simulink model "model_compatible"  (Simulink 7.5)
(part 3 of 4)

      | %<VLF>pu
      | %<angleLF>deg.
      | %<Name>
  bus158 : powerlib/Measurements/Load Flow Bus  LConnTagsString=a  Phases=single  Connectors=on one side  ID=bus158  Vbase=220000  Vref=1  Vangle=0  VLF=1  VLFb=1  VLFc=1  angleLF=0  angleLFb=0  angleLFc=0
      settings: AttributesFormatString=|
      | %<ID>
      | %<Vbase>V
      | %<VLF>pu
      | %<angleLF>deg.
      | %<Name>
  bus159 : powerlib/Measurements/Load Flow Bus  LConnTagsString=a  Phases=single  Connectors=on one side  ID=bus159  Vbase=220000  Vref=1  Vangle=0  VLF=1  VLFb=1  VLFc=1  angleLF=0  angleLFb=0  angleLFc=0
      settings: AttributesFormatString=|
      | %<ID>
      | %<Vbase>V
      | %<VLF>pu
      | %<angleLF>deg.
      | %<Name>
  bus16 : powerlib/Measurements/Load Flow Bus  LConnTagsString=a  Phases=single  Connectors=on one side  ID=bus16  Vbase=220000  Vref=1  Vangle=0  VLF=1  VLFb=1  VLFc=1  angleLF=0  angleLFb=0  angleLFc=0
      settings: AttributesFormatString=|
      | %<ID>
      | %<Vbase>V
      | %<VLF>pu
      | %<angleLF>deg.
      | %<Name>
  bus160 : powerlib/Measurements/Load Flow Bus  LConnTagsString=a  Phases=single  Connectors=on one side  ID=bus160  Vbase=220000  Vref=1  Vangle=0  VLF=1  VLFb=1  VLFc=1  angleLF=0  angleLFb=0  angleLFc=0
      settings: AttributesFormatString=|
      | %<ID>
      | %<Vbase>V
      | %<VLF>pu
      | %<angleLF>deg.
      | %<Name>
  bus161 : powerlib/Measurements/Load Flow Bus  LConnTagsString=a  Phases=single  Connectors=on one side  ID=bus161  Vbase=220000  Vref=1  Vangle=0  VLF=1  VLFb=1  VLFc=1  angleLF=0  angleLFb=0  angleLFc=0
      settings: AttributesFormatString=|
      | %<ID>
      | %<Vbase>V
      | %<VLF>pu
      | %<angleLF>deg.
      | %<Name>
  bus162 : powerlib/Measurements/Load Flow Bus  LConnTagsString=a  Phases=single  Connectors=on one side  ID=bus162  Vbase=220000  Vref=1  Vangle=0  VLF=1  VLFb=1  VLFc=1  angleLF=0  angleLFb=0  angleLFc=0
      settings: AttributesFormatString=|
      | %<ID>
      | %<Vbase>V
      | %<VLF>pu
      | %<angleLF>deg.
      | %<Name>
  bus163 : powerlib/Measurements/Load Flow Bus  LConnTagsString=a  Phases=single  Connectors=on one side  ID=bus163  Vbase=220000  Vref=1  Vangle=0  VLF=1  VLFb=1  VLFc=1  angleLF=0  angleLFb=0  angleLFc=0
      settings: AttributesFormatString=|
      | %<ID>
      | %<Vbase>V
      | %<VLF>pu
      | %<angleLF>deg.
      | %<Name>
  bus164 : powerlib/Measurements/Load Flow Bus  LConnTagsString=a  Phases=single  Connectors=on one side  ID=bus164  Vbase=220000  Vref=1  Vangle=0  VLF=1  VLFb=1  VLFc=1  angleLF=0  angleLFb=0  angleLFc=0
      settings: AttributesFormatString=|
      | %<ID>
      | %<Vbase>V
      | %<VLF>pu
      | %<angleLF>deg.
      | %<Name>
  bus165 : powerlib/Measurements/Load Flow Bus  LConnTagsString=a  Phases=single  Connectors=on one side  ID=bus165  Vbase=220000  Vref=1  Vangle=0  VLF=1  VLFb=1  VLFc=1  angleLF=0  angleLFb=0  angleLFc=0
      settings: AttributesFormatString=|
      | %<ID>
      | %<Vbase>V
      | %<VLF>pu
      | %<angleLF>deg.
      | %<Name>
  bus166 : powerlib/Measurements/Load Flow Bus  LConnTagsString=a  Phases=single  Connectors=on one side  ID=bus166  Vbase=220000  Vref=1  Vangle=0  VLF=1  VLFb=1  VLFc=1  angleLF=0  angleLFb=0  angleLFc=0
      settings: AttributesFormatString=|
      | %<ID>
      | %<Vbase>V
      | %<VLF>pu
      | %<angleLF>deg.
      | %<Name>
  bus167 : powerlib/Measurements/Load Flow Bus  LConnTagsString=a  Phases=single  Connectors=on one side  ID=bus167  Vbase=220000  Vref=1  Vangle=0  VLF=1  VLFb=1  VLFc=1  angleLF=0  angleLFb=0  angleLFc=0
      settings: AttributesFormatString=|
      | %<ID>
      | %<Vbase>V
      | %<VLF>pu
      | %<angleLF>deg.
      | %<Name>
  bus168 : powerlib/Measurements/Load Flow Bus  LConnTagsString=a  Phases=single  Connectors=on one side  ID=bus168  Vbase=220000  Vref=1  Vangle=0  VLF=1  VLFb=1  VLFc=1  angleLF=0  angleLFb=0  angleLFc=0
      settings: AttributesFormatString=|
      | %<ID>
      | %<Vbase>V
      | %<VLF>pu
      | %<angleLF>deg.
      | %<Name>
  bus169 : powerlib/Measurements/Load Flow Bus  LConnTagsString=a  Phases=single  Connectors=on one side  ID=bus169  Vbase=220000  Vref=1  Vangle=0  VLF=1  VLFb=1  VLFc=1  angleLF=0  angleLFb=0  angleLFc=0
      settings: AttributesFormatString=|
      | %<ID>
      | %<Vbase>V
      | %<VLF>pu
      | %<angleLF>deg.
      | %<Name>
  bus17 : powerlib/Measurements/Load Flow Bus  LConnTagsString=a  Phases=single  Connectors=on one side  ID=bus17  Vbase=220000  Vref=1  Vangle=0  VLF=1  VLFb=1  VLFc=1  angleLF=0  angleLFb=0  angleLFc=0
      settings: AttributesFormatString=|
      | %<ID>
      | %<Vbase>V
      | %<VLF>pu
      | %<angleLF>deg.
      | %<Name>
  bus170 : powerlib/Measurements/Load Flow Bus  LConnTagsString=a  Phases=single  Connectors=on one side  ID=bus170  Vbase=220000  Vref=1  Vangle=0  VLF=1  VLFb=1  VLFc=1  angleLF=0  angleLFb=0  angleLFc=0
      settings: AttributesFormatString=|
      | %<ID>
      | %<Vbase>V
      | %<VLF>pu
      | %<angleLF>deg.
      | %<Name>
  bus171 : powerlib/Measurements/Load Flow Bus  LConnTagsString=a  Phases=single  Connectors=on one side  ID=bus171  Vbase=220000  Vref=1  Vangle=0  VLF=1  VLFb=1  VLFc=1  angleLF=0  angleLFb=0  angleLFc=0
      settings: AttributesFormatString=|
      | %<ID>
      | %<Vbase>V
      | %<VLF>pu
      | %<angleLF>deg.
      | %<Name>
  bus172 : powerlib/Measurements/Load Flow Bus  LConnTagsString=a  Phases=single  Connectors=on one side  ID=bus172  Vbase=220000  Vref=1  Vangle=0  VLF=1  VLFb=1  VLFc=1  angleLF=0  angleLFb=0  angleLFc=0
      settings: AttributesFormatString=|
      | %<ID>
      | %<Vbase>V
      | %<VLF>pu
      | %<angleLF>deg.
      | %<Name>
  bus173 : powerlib/Measurements/Load Flow Bus  LConnTagsString=a  Phases=single  Connectors=on one side  ID=bus173  Vbase=220000  Vref=1  Vangle=0  VLF=1  VLFb=1  VLFc=1  angleLF=0  angleLFb=0  angleLFc=0
      settings: AttributesFormatString=|
      | %<ID>
      | %<Vbase>V
      | %<VLF>pu
      | %<angleLF>deg.
      | %<Name>
  bus174 : powerlib/Measurements/Load Flow Bus  LConnTagsString=a  Phases=single  Connectors=on one side  ID=bus174  Vbase=220000  Vref=1  Vangle=0  VLF=1  VLFb=1  VLFc=1  angleLF=0  angleLFb=0  angleLFc=0
      settings: AttributesFormatString=|
      | %<ID>
      | %<Vbase>V
      | %<VLF>pu
      | %<angleLF>deg.
      | %<Name>
  bus175 : powerlib/Measurements/Load Flow Bus  LConnTagsString=a  Phases=single  Connectors=on one side  ID=bus175  Vbase=220000  Vref=1  Vangle=0  VLF=1  VLFb=1  VLFc=1  angleLF=0  angleLFb=0  angleLFc=0
      settings: AttributesFormatString=|
      | %<ID>
      | %<Vbase>V
      | %<VLF>pu
      | %<angleLF>deg.
      | %<Name>
  bus176 : powerlib/Measurements/Load Flow Bus  LConnTagsString=a  Phases=single  Connectors=on one side  ID=bus176  Vbase=220000  Vref=1  Vangle=0  VLF=1  VLFb=1  VLFc=1  angleLF=0  angleLFb=0  angleLFc=0
      settings: AttributesFormatString=|
      | %<ID>
      | %<Vbase>V
      | %<VLF>pu
      | %<angleLF>deg.
      | %<Name>
  bus177 : powerlib/Measurements/Load Flow Bus  LConnTagsString=a  Phases=single  Connectors=on one side  ID=bus177  Vbase=220000  Vref=1  Vangle=0  VLF=1  VLFb=1  VLFc=1  angleLF=0  angleLFb=0  angleLFc=0
      settings: AttributesFormatString=|
      | %<ID>
      | %<Vbase>V
      | %<VLF>pu
      | %<angleLF>deg.
      | %<Name>
  bus178 : powerlib/Measurements/Load Flow Bus  LConnTagsString=a  Phases=single  Connectors=on one side  ID=bus178  Vbase=220000  Vref=1  Vangle=0  VLF=1  VLFb=1  VLFc=1  angleLF=0  angleLFb=0  angleLFc=0
      settings: AttributesFormatString=|
      | %<ID>
      | %<Vbase>V
      | %<VLF>pu
      | %<angleLF>deg.
      | %<Name>
  bus179 : powerlib/Measurements/Load Flow Bus  LConnTagsString=a  Phases=single  Connectors=on one side  ID=bus179  Vbase=220000  Vref=1  Vangle=0  VLF=1  VLFb=1  VLFc=1  angleLF=0  angleLFb=0  angleLFc=0
      settings: AttributesFormatString=|
      | %<ID>
      | %<Vbase>V
      | %<VLF>pu
      | %<angleLF>deg.
      | %<Name>
  bus18 : powerlib/Measurements/Load Flow Bus  LConnTagsString=a  Phases=single  Connectors=on one side  ID=bus18  Vbase=220000  Vref=1  Vangle=0  VLF=1  VLFb=1  VLFc=1  angleLF=0  angleLFb=0  angleLFc=0
      settings: AttributesFormatString=|
      | %<ID>
      | %<Vbase>V
      | %<VLF>pu
      | %<angleLF>deg.
      | %<Name>
  bus180 : powerlib/Measurements/Load Flow Bus  LConnTagsString=a  Phases=single  Connectors=on one side  ID=bus180  Vbase=220000  Vref=1  Vangle=0  VLF=1  VLFb=1  VLFc=1  angleLF=0  angleLFb=0  angleLFc=0
      settings: AttributesFormatString=|
      | %<ID>
      | %<Vbase>V
      | %<VLF>pu
      | %<angleLF>deg.
      | %<Name>
  bus181 : powerlib/Measurements/Load Flow Bus  LConnTagsString=a  Phases=single  Connectors=on one side  ID=bus181  Vbase=220000  Vref=1  Vangle=0  VLF=1  VLFb=1  VLFc=1  angleLF=0  angleLFb=0  angleLFc=0
      settings: AttributesFormatString=|
      | %<ID>
      | %<Vbase>V
      | %<VLF>pu
      | %<angleLF>deg.
      | %<Name>
  bus182 : powerlib/Measurements/Load Flow Bus  LConnTagsString=a  Phases=single  Connectors=on one side  ID=bus182  Vbase=220000  Vref=1  Vangle=0  VLF=1  VLFb=1  VLFc=1  angleLF=0  angleLFb=0  angleLFc=0
      settings: AttributesFormatString=|
      | %<ID>
      | %<Vbase>V
      | %<VLF>pu
      | %<angleLF>deg.
      | %<Name>
  bus183 : powerlib/Measurements/Load Flow Bus  LConnTagsString=a  Phases=single  Connectors=on one side  ID=bus183  Vbase=220000  Vref=1  Vangle=0  VLF=1  VLFb=1  VLFc=1  angleLF=0  angleLFb=0  angleLFc=0
      settings: AttributesFormatString=|
      | %<ID>
      | %<Vbase>V
      | %<VLF>pu
      | %<angleLF>deg.
      | %<Name>
  bus184 : powerlib/Measurements/Load Flow Bus  LConnTagsString=a  Phases=single  Connectors=on one side  ID=bus184  Vbase=220000  Vref=1  Vangle=0  VLF=1  VLFb=1  VLFc=1  angleLF=0  angleLFb=0  angleLFc=0
      settings: AttributesFormatString=|
      | %<ID>
      | %<Vbase>V
      | %<VLF>pu
      | %<angleLF>deg.
      | %<Name>
  bus185 : powerlib/Measurements/Load Flow Bus  LConnTagsString=a  Phases=single  Connectors=on one side  ID=bus185  Vbase=220000  Vref=1  Vangle=0  VLF=1  VLFb=1  VLFc=1  angleLF=0  angleLFb=0  angleLFc=0
      settings: AttributesFormatString=|
      | %<ID>
      | %<Vbase>V
      | %<VLF>pu
      | %<angleLF>deg.
      | %<Name>
  bus186 : powerlib/Measurements/Load Flow Bus  LConnTagsString=a  Phases=single  Connectors=on one side  ID=bus186  Vbase=220000  Vref=1  Vangle=0  VLF=1  VLFb=1  VLFc=1  angleLF=0  angleLFb=0  angleLFc=0
      settings: AttributesFormatString=|
      | %<ID>
      | %<Vbase>V
      | %<VLF>pu
      | %<angleLF>deg.
      | %<Name>
  bus187 : powerlib/Measurements/Load Flow Bus  LConnTagsString=a  Phases=single  Connectors=on one side  ID=bus187  Vbase=220000  Vref=1  Vangle=0  VLF=1  VLFb=1  VLFc=1  angleLF=0  angleLFb=0  angleLFc=0
      settings: AttributesFormatString=|
      | %<ID>
      | %<Vbase>V
      | %<VLF>pu
      | %<angleLF>deg.
      | %<Name>
  bus188 : powerlib/Measurements/Load Flow Bus  LConnTagsString=a  Phases=single  Connectors=on one side  ID=bus188  Vbase=220000  Vref=1  Vangle=0  VLF=1  VLFb=1  VLFc=1  angleLF=0  angleLFb=0  angleLFc=0
      settings: AttributesFormatString=|
      | %<ID>
      | %<Vbase>V
      | %<VLF>pu
      | %<angleLF>deg.
      | %<Name>
  bus189 : powerlib/Measurements/Load Flow Bus  LConnTagsString=a  Phases=single  Connectors=on one side  ID=bus189  Vbase=220000  Vref=1  Vangle=0  VLF=1  VLFb=1  VLFc=1  angleLF=0  angleLFb=0  angleLFc=0
      settings: AttributesFormatString=|
      | %<ID>
      | %<Vbase>V
      | %<VLF>pu
      | %<angleLF>deg.
      | %<Name>
  bus19 : powerlib/Measurements/Load Flow Bus  LConnTagsString=a  Phases=single  Connectors=on one side  ID=bus19  Vbase=220000  Vref=1  Vangle=0  VLF=1  VLFb=1  VLFc=1  angleLF=0  angleLFb=0  angleLFc=0
      settings: AttributesFormatString=|
      | %<ID>
      | %<Vbase>V
      | %<VLF>pu
      | %<angleLF>deg.
      | %<Name>
  bus190 : powerlib/Measurements/Load Flow Bus  LConnTagsString=a  Phases=single  Connectors=on one side  ID=bus190  Vbase=220000  Vref=1  Vangle=0  VLF=1  VLFb=1  VLFc=1  angleLF=0  angleLFb=0  angleLFc=0
      settings: AttributesFormatString=|
      | %<ID>
      | %<Vbase>V
      | %<VLF>pu
      | %<angleLF>deg.
      | %<Name>
  bus191 : powerlib/Measurements/Load Flow Bus  LConnTagsString=a  Phases=single  Connectors=on one side  ID=bus191  Vbase=220000  Vref=1  Vangle=0  VLF=1  VLFb=1  VLFc=1  angleLF=0  angleLFb=0  angleLFc=0
      settings: AttributesFormatString=|
      | %<ID>
      | %<Vbase>V
      | %<VLF>pu
      | %<angleLF>deg.
      | %<Name>
  bus192 : powerlib/Measurements/Load Flow Bus  LConnTagsString=a  Phases=single  Connectors=on one side  ID=bus192  Vbase=220000  Vref=1  Vangle=0  VLF=1  VLFb=1  VLFc=1  angleLF=0  angleLFb=0  angleLFc=0
      settings: AttributesFormatString=|
      | %<ID>
      | %<Vbase>V
      | %<VLF>pu
      | %<angleLF>deg.
      | %<Name>
  bus193 : powerlib/Measurements/Load Flow Bus  LConnTagsString=a  Phases=single  Connectors=on one side  ID=bus193  Vbase=220000  Vref=1  Vangle=0  VLF=1  VLFb=1  VLFc=1  angleLF=0  angleLFb=0  angleLFc=0
      settings: AttributesFormatString=|
      | %<ID>
      | %<Vbase>V
      | %<VLF>pu
      | %<angleLF>deg.
      | %<Name>
  bus194 : powerlib/Measurements/Load Flow Bus  LConnTagsString=a  Phases=single  Connectors=on one side  ID=bus194  Vbase=220000  Vref=1  Vangle=0  VLF=1  VLFb=1  VLFc=1  angleLF=0  angleLFb=0  angleLFc=0
      settings: AttributesFormatString=|
      | %<ID>
      | %<Vbase>V
      | %<VLF>pu
      | %<angleLF>deg.
      | %<Name>
  bus195 : powerlib/Measurements/Load Flow Bus  LConnTagsString=a  Phases=single  Connectors=on one side  ID=bus195  Vbase=220000  Vref=1  Vangle=0  VLF=1  VLFb=1  VLFc=1  angleLF=0  angleLFb=0  angleLFc=0
      settings: AttributesFormatString=|
      | %<ID>
      | %<Vbase>V
      | %<VLF>pu
      | %<angleLF>deg.
      | %<Name>
  bus196 : powerlib/Measurements/Load Flow Bus  LConnTagsString=a  Phases=single  Connectors=on one side  ID=bus196  Vbase=220000  Vref=1  Vangle=0  VLF=1  VLFb=1  VLFc=1  angleLF=0  angleLFb=0  angleLFc=0
      settings: AttributesFormatString=|
      | %<ID>
      | %<Vbase>V
      | %<VLF>pu
      | %<angleLF>deg.
      | %<Name>
  bus197 : powerlib/Measurements/Load Flow Bus  LConnTagsString=a  Phases=single  Connectors=on one side  ID=bus197  Vbase=220000  Vref=1  Vangle=0  VLF=1  VLFb=1  VLFc=1  angleLF=0  angleLFb=0  angleLFc=0
      settings: AttributesFormatString=|
      | %<ID>
      | %<Vbase>V
      | %<VLF>pu
      | %<angleLF>deg.
      | %<Name>
  bus198 : powerlib/Measurements/Load Flow Bus  LConnTagsString=a  Phases=single  Connectors=on one side  ID=bus198  Vbase=220000  Vref=1  Vangle=0  VLF=1  VLFb=1  VLFc=1  angleLF=0  angleLFb=0  angleLFc=0
      settings: AttributesFormatString=|
      | %<ID>
      | %<Vbase>V
      | %<VLF>pu
      | %<angleLF>deg.
      | %<Name>
  bus199 : powerlib/Measurements/Load Flow Bus  LConnTagsString=a  Phases=single  Connectors=on one side  ID=bus199  Vbase=220000  Vref=1  Vangle=0  VLF=1  VLFb=1  VLFc=1  angleLF=0  angleLFb=0  angleLFc=0
      settings: AttributesFormatString=|
      | %<ID>
      | %<Vbase>V
      | %<VLF>pu
      | %<angleLF>deg.
      | %<Name>
  bus2 : powerlib/Measurements/Load Flow Bus  LConnTagsString=a  Phases=single  Connectors=on one side  ID=bus2  Vbase=220000  Vref=1  Vangle=0  VLF=1  VLFb=1  VLFc=1  angleLF=0  angleLFb=0  angleLFc=0
      settings: AttributesFormatString=|
      | %<ID>
      | %<Vbase>V
      | %<VLF>pu
      | %<angleLF>deg.
      | %<Name>
  bus20 : powerlib/Measurements/Load Flow Bus  LConnTagsString=a  Phases=single  Connectors=on one side  ID=bus20  Vbase=220000  Vref=1  Vangle=0  VLF=1  VLFb=1  VLFc=1  angleLF=0  angleLFb=0  angleLFc=0
      settings: AttributesFormatString=|
      | %<ID>
      | %<Vbase>V
      | %<VLF>pu
      | %<angleLF>deg.
      | %<Name>
  bus200 : powerlib/Measurements/Load Flow Bus  LConnTagsString=a  Phases=single  Connectors=on one side  ID=bus200  Vbase=220000  Vref=1  Vangle=0  VLF=1  VLFb=1  VLFc=1  angleLF=0  angleLFb=0  angleLFc=0
      settings: AttributesFormatString=|
      | %<ID>
      | %<Vbase>V
      | %<VLF>pu
      | %<angleLF>deg.
      | %<Name>
  bus201 : powerlib/Measurements/Load Flow Bus  LConnTagsString=a  Phases=single  Connectors=on one side  ID=bus201  Vbase=220000  Vref=1  Vangle=0  VLF=1  VLFb=1  VLFc=1  angleLF=0  angleLFb=0  angleLFc=0
      settings: AttributesFormatString=|
      | %<ID>
      | %<Vbase>V
      | %<VLF>pu
      | %<angleLF>deg.
      | %<Name>
  bus202 : powerlib/Measurements/Load Flow Bus  LConnTagsString=a  Phases=single  Connectors=on one side  ID=bus202  Vbase=220000  Vref=1  Vangle=0  VLF=1  VLFb=1  VLFc=1  angleLF=0  angleLFb=0  angleLFc=0
      settings: AttributesFormatString=|
      | %<ID>
      | %<Vbase>V
      | %<VLF>pu
      | %<angleLF>deg.
      | %<Name>
  bus203 : powerlib/Measurements/Load Flow Bus  LConnTagsString=a  Phases=single  Connectors=on one side  ID=bus203  Vbase=220000  Vref=1  Vangle=0  VLF=1  VLFb=1  VLFc=1  angleLF=0  angleLFb=0  angleLFc=0
      settings: AttributesFormatString=|
      | %<ID>
      | %<Vbase>V
      | %<VLF>pu
      | %<angleLF>deg.
      | %<Name>
  bus204 : powerlib/Measurements/Load Flow Bus  LConnTagsString=a  Phases=single  Connectors=on one side  ID=bus204  Vbase=220000  Vref=1  Vangle=0  VLF=1  VLFb=1  VLFc=1  angleLF=0  angleLFb=0  angleLFc=0
      settings: AttributesFormatString=|
      | %<ID>
      | %<Vbase>V
      | %<VLF>pu
      | %<angleLF>deg.
      | %<Name>
  bus205 : powerlib/Measurements/Load Flow Bus  LConnTagsString=a  Phases=single  Connectors=on one side  ID=bus205  Vbase=220000  Vref=1  Vangle=0  VLF=1  VLFb=1  VLFc=1  angleLF=0  angleLFb=0  angleLFc=0
      settings: AttributesFormatString=|
      | %<ID>
      | %<Vbase>V
      | %<VLF>pu
      | %<angleLF>deg.
      | %<Name>
  bus206 : powerlib/Measurements/Load Flow Bus  LConnTagsString=a  Phases=single  Connectors=on one side  ID=bus206  Vbase=220000  Vref=1  Vangle=0  VLF=1  VLFb=1  VLFc=1  angleLF=0  angleLFb=0  angleLFc=0
      settings: AttributesFormatString=|
      | %<ID>
      | %<Vbase>V
      | %<VLF>pu
      | %<angleLF>deg.
      | %<Name>
  bus207 : powerlib/Measurements/Load Flow Bus  LConnTagsString=a  Phases=single  Connectors=on one side  ID=bus207  Vbase=220000  Vref=1  Vangle=0  VLF=1  VLFb=1  VLFc=1  angleLF=0  angleLFb=0  angleLFc=0
      settings: AttributesFormatString=|
      | %<ID>
      | %<Vbase>V
      | %<VLF>pu
      | %<angleLF>deg.
      | %<Name>
  bus208 : powerlib/Measurements/Load Flow Bus  LConnTagsString=a  Phases=single  Connectors=on one side  ID=bus208  Vbase=220000  Vref=1  Vangle=0  VLF=1  VLFb=1  VLFc=1  angleLF=0  angleLFb=0  angleLFc=0
      settings: AttributesFormatString=|
      | %<ID>
      | %<Vbase>V
      | %<VLF>pu
      | %<angleLF>deg.
      | %<Name>
  bus209 : powerlib/Measurements/Load Flow Bus  LConnTagsString=a  Phases=single  Connectors=on one side  ID=bus209  Vbase=220000  Vref=1  Vangle=0  VLF=1  VLFb=1  VLFc=1  angleLF=0  angleLFb=0  angleLFc=0
      settings: AttributesFormatString=|
      | %<ID>
      | %<Vbase>V
      | %<VLF>pu
      | %<angleLF>deg.
      | %<Name>
  bus21 : powerlib/Measurements/Load Flow Bus  LConnTagsString=a  Phases=single  Connectors=on one side  ID=bus21  Vbase=220000  Vref=1  Vangle=0  VLF=1  VLFb=1  VLFc=1  angleLF=0  angleLFb=0  angleLFc=0
      settings: AttributesFormatString=|
      | %<ID>
      | %<Vbase>V
      | %<VLF>pu
      | %<angleLF>deg.
      | %<Name>
  bus210 : powerlib/Measurements/Load Flow Bus  LConnTagsString=a  Phases=single  Connectors=on one side  ID=bus210  Vbase=220000  Vref=1  Vangle=0  VLF=1  VLFb=1  VLFc=1  angleLF=0  angleLFb=0  angleLFc=0
      settings: AttributesFormatString=|
      | %<ID>
      | %<Vbase>V
      | %<VLF>pu
      | %<angleLF>deg.
      | %<Name>
  bus211 : powerlib/Measurements/Load Flow Bus  LConnTagsString=a  Phases=single  Connectors=on one side  ID=bus211  Vbase=220000  Vref=1  Vangle=0  VLF=1  VLFb=1  VLFc=1  angleLF=0  angleLFb=0  angleLFc=0
      settings: AttributesFormatString=|
      | %<ID>
      | %<Vbase>V
      | %<VLF>pu
      | %<angleLF>deg.
      | %<Name>
  bus212 : powerlib/Measurements/Load Flow Bus  LConnTagsString=a  Phases=single  Connectors=on one side  ID=bus212  Vbase=220000  Vref=1  Vangle=0  VLF=1  VLFb=1  VLFc=1  angleLF=0  angleLFb=0  angleLFc=0
      settings: AttributesFormatString=|
      | %<ID>
      | %<Vbase>V
      | %<VLF>pu
      | %<angleLF>deg.
      | %<Name>
  bus213 : powerlib/Measurements/Load Flow Bus  LConnTagsString=a  Phases=single  Connectors=on one side  ID=bus213  Vbase=220000  Vref=1  Vangle=0  VLF=1  VLFb=1  VLFc=1  angleLF=0  angleLFb=0  angleLFc=0
      settings: AttributesFormatString=|
      | %<ID>
      | %<Vbase>V
      | %<VLF>pu
      | %<angleLF>deg.
      | %<Name>
  bus214 : powerlib/Measurements/Load Flow Bus  LConnTagsString=a  Phases=single  Connectors=on one side  ID=bus214  Vbase=220000  Vref=1  Vangle=0  VLF=1  VLFb=1  VLFc=1  angleLF=0  angleLFb=0  angleLFc=0
      settings: AttributesFormatString=|
      | %<ID>
      | %<Vbase>V
      | %<VLF>pu
      | %<angleLF>deg.
      | %<Name>
  bus215 : powerlib/Measurements/Load Flow Bus  LConnTagsString=a  Phases=single  Connectors=on one side  ID=bus215  Vbase=220000  Vref=1  Vangle=0  VLF=1  VLFb=1  VLFc=1  angleLF=0  angleLFb=0  angleLFc=0
      settings: AttributesFormatString=|
      | %<ID>
      | %<Vbase>V
      | %<VLF>pu
      | %<angleLF>deg.
      | %<Name>
  bus216 : powerlib/Measurements/Load Flow Bus  LConnTagsString=a  Phases=single  Connectors=on one side  ID=bus216  Vbase=220000  Vref=1  Vangle=0  VLF=1  VLFb=1  VLFc=1  angleLF=0  angleLFb=0  angleLFc=0
      settings: AttributesFormatString=|
      | %<ID>
      | %<Vbase>V
      | %<VLF>pu
      | %<angleLF>deg.
      | %<Name>
  bus217 : powerlib/Measurements/Load Flow Bus  LConnTagsString=a  Phases=single  Connectors=on one side  ID=bus217  Vbase=220000  Vref=1  Vangle=0  VLF=1  VLFb=1  VLFc=1  angleLF=0  angleLFb=0  angleLFc=0
      settings: AttributesFormatString=|
      | %<ID>
      | %<Vbase>V
      | %<VLF>pu
      | %<angleLF>deg.
      | %<Name>
  bus218 : powerlib/Measurements/Load Flow Bus  LConnTagsString=a  Phases=single  Connectors=on one side  ID=bus218  Vbase=220000  Vref=1  Vangle=0  VLF=1  VLFb=1  VLFc=1  angleLF=0  angleLFb=0  angleLFc=0
      settings: AttributesFormatString=|
      | %<ID>
      | %<Vbase>V
      | %<VLF>pu
      | %<angleLF>deg.
      | %<Name>
  bus219 : powerlib/Measurements/Load Flow Bus  LConnTagsString=a  Phases=single  Connectors=on one side  ID=bus219  Vbase=220000  Vref=1  Vangle=0  VLF=1  VLFb=1  VLFc=1  angleLF=0  angleLFb=0  angleLFc=0
      settings: AttributesFormatString=|
      | %<ID>
      | %<Vbase>V
      | %<VLF>pu
      | %<angleLF>deg.
      | %<Name>
  bus22 : powerlib/Measurements/Load Flow Bus  LConnTagsString=a  Phases=single  Connectors=on one side  ID=bus22  Vbase=220000  Vref=1  Vangle=0  VLF=1  VLFb=1  VLFc=1  angleLF=0  angleLFb=0  angleLFc=0
      settings: AttributesFormatString=|
      | %<ID>
      | %<Vbase>V
      | %<VLF>pu
      | %<angleLF>deg.
      | %<Name>
  bus220 : powerlib/Measurements/Load Flow Bus  LConnTagsString=a  Phases=single  Connectors=on one side  ID=bus220  Vbase=220000  Vref=1  Vangle=0  VLF=1  VLFb=1  VLFc=1  angleLF=0  angleLFb=0  angleLFc=0
      settings: AttributesFormatString=|
      | %<ID>
      | %<Vbase>V
      | %<VLF>pu
      | %<angleLF>deg.
      | %<Name>
  bus221 : powerlib/Measurements/Load Flow Bus  LConnTagsString=a  Phases=single  Connectors=on one side  ID=bus221  Vbase=220000  Vref=1  Vangle=0  VLF=1  VLFb=1  VLFc=1  angleLF=0  angleLFb=0  angleLFc=0
      settings: AttributesFormatString=|
      | %<ID>
      | %<Vbase>V
      | %<VLF>pu
      | %<angleLF>deg.
      | %<Name>
  bus222 : powerlib/Measurements/Load Flow Bus  LConnTagsString=a  Phases=single  Connectors=on one side  ID=bus222  Vbase=220000  Vref=1  Vangle=0  VLF=1  VLFb=1  VLFc=1  angleLF=0  angleLFb=0  angleLFc=0
      settings: AttributesFormatString=|
      | %<ID>
      | %<Vbase>V
      | %<VLF>pu
      | %<angleLF>deg.
      | %<Name>
  bus223 : powerlib/Measurements/Load Flow Bus  LConnTagsString=a  Phases=single  Connectors=on one side  ID=bus223  Vbase=220000  Vref=1  Vangle=0  VLF=1  VLFb=1  VLFc=1  angleLF=0  angleLFb=0  angleLFc=0
      settings: AttributesFormatString=|
      | %<ID>
      | %<Vbase>V
      | %<VLF>pu
      | %<angleLF>deg.
      | %<Name>
  bus224 : powerlib/Measurements/Load Flow Bus  LConnTagsString=a  Phases=single  Connectors=on one side  ID=bus224  Vbase=220000  Vref=1  Vangle=0  VLF=1  VLFb=1  VLFc=1  angleLF=0  angleLFb=0  angleLFc=0
      settings: AttributesFormatString=|
      | %<ID>
      | %<Vbase>V
      | %<VLF>pu
      | %<angleLF>deg.
      | %<Name>
  bus225 : powerlib/Measurements/Load Flow Bus  LConnTagsString=a  Phases=single  Connectors=on one side  ID=bus225  Vbase=220000  Vref=1  Vangle=0  VLF=1  VLFb=1  VLFc=1  angleLF=0  angleLFb=0  angleLFc=0
      settings: AttributesFormatString=|
      | %<ID>
      | %<Vbase>V
      | %<VLF>pu
      | %<angleLF>deg.
      | %<Name>
  bus226 : powerlib/Measurements/Load Flow Bus  LConnTagsString=a  Phases=single  Connectors=on one side  ID=bus226  Vbase=220000  Vref=1  Vangle=0  VLF=1  VLFb=1  VLFc=1  angleLF=0  angleLFb=0  angleLFc=0
      settings: AttributesFormatString=|
      | %<ID>
      | %<Vbase>V
      | %<VLF>pu
      | %<angleLF>deg.
      | %<Name>
  bus227 : powerlib/Measurements/Load Flow Bus  LConnTagsString=a  Phases=single  Connectors=on one side  ID=bus227  Vbase=400000  Vref=1  Vangle=0  VLF=1  VLFb=1  VLFc=1  angleLF=0  angleLFb=0  angleLFc=0
      settings: AttributesFormatString=|
      | %<ID>
      | %<Vbase>V
      | %<VLF>pu
      | %<angleLF>deg.
      | %<Name>
  bus228 : powerlib/Measurements/Load Flow Bus  LConnTagsString=a  Phases=single  Connectors=on one side  ID=bus228  Vbase=400000  Vref=1  Vangle=0  VLF=1  VLFb=1  VLFc=1  angleLF=0  angleLFb=0  angleLFc=0
      settings: AttributesFormatString=|
      | %<ID>
      | %<Vbase>V
      | %<VLF>pu
      | %<angleLF>deg.
      | %<Name>
  bus229 : powerlib/Measurements/Load Flow Bus  LConnTagsString=a  Phases=single  Connectors=on one side  ID=bus229  Vbase=400000  Vref=1  Vangle=0  VLF=1  VLFb=1  VLFc=1  angleLF=0  angleLFb=0  angleLFc=0
      settings: AttributesFormatString=|
      | %<ID>
      | %<Vbase>V
      | %<VLF>pu
      | %<angleLF>deg.
      | %<Name>
  bus23 : powerlib/Measurements/Load Flow Bus  LConnTagsString=a  Phases=single  Connectors=on one side  ID=bus23  Vbase=220000  Vref=1  Vangle=0  VLF=1  VLFb=1  VLFc=1  angleLF=0  angleLFb=0  angleLFc=0
      settings: AttributesFormatString=|
      | %<ID>
      | %<Vbase>V
      | %<VLF>pu
      | %<angleLF>deg.
      | %<Name>
  bus230 : powerlib/Measurements/Load Flow Bus  LConnTagsString=a  Phases=single  Connectors=on one side  ID=bus230  Vbase=400000  Vref=1  Vangle=0  VLF=1  VLFb=1  VLFc=1  angleLF=0  angleLFb=0  angleLFc=0
      settings: AttributesFormatString=|
      | %<ID>
      | %<Vbase>V
      | %<VLF>pu
      | %<angleLF>deg.
      | %<Name>
  bus231 : powerlib/Measurements/Load Flow Bus  LConnTagsString=a  Phases=single  Connectors=on one side  ID=bus231  Vbase=400000  Vref=1  Vangle=0  VLF=1  VLFb=1  VLFc=1  angleLF=0  angleLFb=0  angleLFc=0
      settings: AttributesFormatString=|
      | %<ID>
      | %<Vbase>V
      | %<VLF>pu
      | %<angleLF>deg.
      | %<Name>
  bus232 : powerlib/Measurements/Load Flow Bus  LConnTagsString=a  Phases=single  Connectors=on one side  ID=bus232  Vbase=400000  Vref=1  Vangle=0  VLF=1  VLFb=1  VLFc=1  angleLF=0  angleLFb=0  angleLFc=0
      settings: AttributesFormatString=|
      | %<ID>
      | %<Vbase>V
      | %<VLF>pu
      | %<angleLF>deg.
      | %<Name>
  bus233 : powerlib/Measurements/Load Flow Bus  LConnTagsString=a  Phases=single  Connectors=on one side  ID=bus233  Vbase=400000  Vref=1  Vangle=0  VLF=1  VLFb=1  VLFc=1  angleLF=0  angleLFb=0  angleLFc=0
      settings: AttributesFormatString=|
      | %<ID>
      | %<Vbase>V
      | %<VLF>pu
      | %<angleLF>deg.
      | %<Name>
  bus234 : powerlib/Measurements/Load Flow Bus  LConnTagsString=a  Phases=single  Connectors=on one side  ID=bus234  Vbase=400000  Vref=1  Vangle=0  VLF=1  VLFb=1  VLFc=1  angleLF=0  angleLFb=0  angleLFc=0
      settings: AttributesFormatString=|
      | %<ID>
      | %<Vbase>V
      | %<VLF>pu
      | %<angleLF>deg.
      | %<Name>
  bus235 : powerlib/Measurements/Load Flow Bus  LConnTagsString=a  Phases=single  Connectors=on one side  ID=bus235  Vbase=400000  Vref=1  Vangle=0  VLF=1  VLFb=1  VLFc=1  angleLF=0  angleLFb=0  angleLFc=0
      settings: AttributesFormatString=|
      | %<ID>
      | %<Vbase>V
      | %<VLF>pu
      | %<angleLF>deg.
      | %<Name>
  bus236 : powerlib/Measurements/Load Flow Bus  LConnTagsString=a  Phases=single  Connectors=on one side  ID=bus236  Vbase=400000  Vref=1  Vangle=0  VLF=1  VLFb=1  VLFc=1  angleLF=0  angleLFb=0  angleLFc=0
      settings: AttributesFormatString=|
      | %<ID>
      | %<Vbase>V
      | %<VLF>pu
      | %<angleLF>deg.
      | %<Name>
  bus237 : powerlib/Measurements/Load Flow Bus  LConnTagsString=a  Phases=single  Connectors=on one side  ID=bus237  Vbase=400000  Vref=1  Vangle=0  VLF=1  VLFb=1  VLFc=1  angleLF=0  angleLFb=0  angleLFc=0
      settings: AttributesFormatString=|
      | %<ID>
      | %<Vbase>V
      | %<VLF>pu
      | %<angleLF>deg.
      | %<Name>
  bus238 : powerlib/Measurements/Load Flow Bus  LConnTagsString=a  Phases=single  Connectors=on one side  ID=bus238  Vbase=400000  Vref=1  Vangle=0  VLF=1  VLFb=1  VLFc=1  angleLF=0  angleLFb=0  angleLFc=0
      settings: AttributesFormatString=|
      | %<ID>
      | %<Vbase>V
      | %<VLF>pu
      | %<angleLF>deg.
      | %<Name>
  bus239 : powerlib/Measurements/Load Flow Bus  LConnTagsString=a  Phases=single  Connectors=on one side  ID=bus239  Vbase=400000  Vref=1  Vangle=0  VLF=1  VLFb=1  VLFc=1  angleLF=0  angleLFb=0  angleLFc=0
      settings: AttributesFormatString=|
      | %<ID>
      | %<Vbase>V
      | %<VLF>pu
      | %<angleLF>deg.
      | %<Name>
  bus24 : powerlib/Measurements/Load Flow Bus  LConnTagsString=a  Phases=single  Connectors=on one side  ID=bus24  Vbase=220000  Vref=1  Vangle=0  VLF=1  VLFb=1  VLFc=1  angleLF=0  angleLFb=0  angleLFc=0
      settings: AttributesFormatString=|
      | %<ID>
      | %<Vbase>V
      | %<VLF>pu
      | %<angleLF>deg.
      | %<Name>
  bus240 : powerlib/Measurements/Load Flow Bus  LConnTagsString=a  Phases=single  Connectors=on one side  ID=bus240  Vbase=400000  Vref=1  Vangle=0  VLF=1  VLFb=1  VLFc=1  angleLF=0  angleLFb=0  angleLFc=0
      settings: AttributesFormatString=|
      | %<ID>
      | %<Vbase>V
      | %<VLF>pu
      | %<angleLF>deg.
      | %<Name>
  bus241 : powerlib/Measurements/Load Flow Bus  LConnTagsString=a  Phases=single  Connectors=on one side  ID=bus241  Vbase=400000  Vref=1  Vangle=0  VLF=1  VLFb=1  VLFc=1  angleLF=0  angleLFb=0  angleLFc=0
      settings: AttributesFormatString=|
      | %<ID>
      | %<Vbase>V
      | %<VLF>pu
      | %<angleLF>deg.
      | %<Name>
  bus242 : powerlib/Measurements/Load Flow Bus  LConnTagsString=a  Phases=single  Connectors=on one side  ID=bus242  Vbase=400000  Vref=1  Vangle=0  VLF=1  VLFb=1  VLFc=1  angleLF=0  angleLFb=0  angleLFc=0
      settings: AttributesFormatString=|
      | %<ID>
      | %<Vbase>V
      | %<VLF>pu
      | %<angleLF>deg.
      | %<Name>
  bus243 : powerlib/Measurements/Load Flow Bus  LConnTagsString=a  Phases=single  Connectors=on one side  ID=bus243  Vbase=400000  Vref=1  Vangle=0  VLF=1  VLFb=1  VLFc=1  angleLF=0  angleLFb=0  angleLFc=0
      settings: AttributesFormatString=|
      | %<ID>
      | %<Vbase>V
      | %<VLF>pu
      | %<angleLF>deg.
      | %<Name>
  bus244 : powerlib/Measurements/Load Flow Bus  LConnTagsString=a  Phases=single  Connectors=on one side  ID=bus244  Vbase=400000  Vref=1  Vangle=0  VLF=1  VLFb=1  VLFc=1  angleLF=0  angleLFb=0  angleLFc=0
      settings: AttributesFormatString=|
      | %<ID>
      | %<Vbase>V
      | %<VLF>pu
      | %<angleLF>deg.
      | %<Name>
  bus245 : powerlib/Measurements/Load Flow Bus  LConnTagsString=a  Phases=single  Connectors=on one side  ID=bus245  Vbase=400000  Vref=1  Vangle=0  VLF=1  VLFb=1  VLFc=1  angleLF=0  angleLFb=0  angleLFc=0
      settings: AttributesFormatString=|
      | %<ID>
      | %<Vbase>V
      | %<VLF>pu
      | %<angleLF>deg.
      | %<Name>
  bus246 : powerlib/Measurements/Load Flow Bus  LConnTagsString=a  Phases=single  Connectors=on one side  ID=bus246  Vbase=400000  Vref=1  Vangle=0  VLF=1  VLFb=1  VLFc=1  angleLF=0  angleLFb=0  angleLFc=0
      settings: AttributesFormatString=|
      | %<ID>
      | %<Vbase>V
      | %<VLF>pu
      | %<angleLF>deg.
      | %<Name>
  bus247 : powerlib/Measurements/Load Flow Bus  LConnTagsString=a  Phases=single  Connectors=on one side  ID=bus247  Vbase=400000  Vref=1  Vangle=0  VLF=1  VLFb=1  VLFc=1  angleLF=0  angleLFb=0  angleLFc=0
      settings: AttributesFormatString=|
      | %<ID>
      | %<Vbase>V
      | %<VLF>pu
      | %<angleLF>deg.
      | %<Name>
  bus248 : powerlib/Measurements/Load Flow Bus  LConnTagsString=a  Phases=single  Connectors=on one side  ID=bus248  Vbase=400000  Vref=1  Vangle=0  VLF=1  VLFb=1  VLFc=1  angleLF=0  angleLFb=0  angleLFc=0
      settings: AttributesFormatString=|
      | %<ID>
      | %<Vbase>V
      | %<VLF>pu
      | %<angleLF>deg.
      | %<Name>
  bus249 : powerlib/Measurements/Load Flow Bus  LConnTagsString=a  Phases=single  Connectors=on one side  ID=bus249  Vbase=400000  Vref=1  Vangle=0  VLF=1  VLFb=1  VLFc=1  angleLF=0  angleLFb=0  angleLFc=0
      settings: AttributesFormatString=|
      | %<ID>
      | %<Vbase>V
      | %<VLF>pu
      | %<angleLF>deg.
      | %<Name>
  bus25 : powerlib/Measurements/Load Flow Bus  LConnTagsString=a  Phases=single  Connectors=on one side  ID=bus25  Vbase=220000  Vref=1  Vangle=0  VLF=1  VLFb=1  VLFc=1  angleLF=0  angleLFb=0  angleLFc=0
      settings: AttributesFormatString=|
      | %<ID>
      | %<Vbase>V
      | %<VLF>pu
      | %<angleLF>deg.
      | %<Name>
  bus250 : powerlib/Measurements/Load Flow Bus  LConnTagsString=a  Phases=single  Connectors=on one side  ID=bus250  Vbase=400000  Vref=1  Vangle=0  VLF=1  VLFb=1  VLFc=1  angleLF=0  angleLFb=0  angleLFc=0
      settings: AttributesFormatString=|
      | %<ID>
      | %<Vbase>V
      | %<VLF>pu
      | %<angleLF>deg.
      | %<Name>
  bus251 : powerlib/Measurements/Load Flow Bus  LConnTagsString=a  Phases=single  Connectors=on one side  ID=bus251  Vbase=400000  Vref=1  Vangle=0  VLF=1  VLFb=1  VLFc=1  angleLF=0  angleLFb=0  angleLFc=0
      settings: AttributesFormatString=|
      | %<ID>
      | %<Vbase>V
      | %<VLF>pu
      | %<angleLF>deg.
      | %<Name>
  bus252 : powerlib/Measurements/Load Flow Bus  LConnTagsString=a  Phases=single  Connectors=on one side  ID=bus252  Vbase=400000  Vref=1  Vangle=0  VLF=1  VLFb=1  VLFc=1  angleLF=0  angleLFb=0  angleLFc=0
      settings: AttributesFormatString=|
      | %<ID>
      | %<Vbase>V
      | %<VLF>pu
      | %<angleLF>deg.
      | %<Name>
  bus253 : powerlib/Measurements/Load Flow Bus  LConnTagsString=a  Phases=single  Connectors=on one side  ID=bus253  Vbase=400000  Vref=1  Vangle=0  VLF=1  VLFb=1  VLFc=1  angleLF=0  angleLFb=0  angleLFc=0
      settings: AttributesFormatString=|
      | %<ID>
      | %<Vbase>V
      | %<VLF>pu
      | %<angleLF>deg.
      | %<Name>
  bus254 : powerlib/Measurements/Load Flow Bus  LConnTagsString=a  Phases=single  Connectors=on one side  ID=bus254  Vbase=400000  Vref=1  Vangle=0  VLF=1  VLFb=1  VLFc=1  angleLF=0  angleLFb=0  angleLFc=0
      settings: AttributesFormatString=|
      | %<ID>
      | %<Vbase>V
      | %<VLF>pu
      | %<angleLF>deg.
      | %<Name>
  bus255 : powerlib/Measurements/Load Flow Bus  LConnTagsString=a  Phases=single  Connectors=on one side  ID=bus255  Vbase=400000  Vref=1  Vangle=0  VLF=1  VLFb=1  VLFc=1  angleLF=0  angleLFb=0  angleLFc=0
      settings: AttributesFormatString=|
      | %<ID>
      | %<Vbase>V
      | %<VLF>pu
      | %<angleLF>deg.
      | %<Name>
  bus256 : powerlib/Measurements/Load Flow Bus  LConnTagsString=a  Phases=single  Connectors=on one side  ID=bus256  Vbase=400000  Vref=1  Vangle=0  VLF=1  VLFb=1  VLFc=1  angleLF=0  angleLFb=0  angleLFc=0
      settings: AttributesFormatString=|
      | %<ID>
      | %<Vbase>V
      | %<VLF>pu
      | %<angleLF>deg.
      | %<Name>
  bus26 : powerlib/Measurements/Load Flow Bus  LConnTagsString=a  Phases=single  Connectors=on one side  ID=bus26  Vbase=220000  Vref=1  Vangle=0  VLF=1  VLFb=1  VLFc=1  angleLF=0  angleLFb=0  angleLFc=0
      settings: AttributesFormatString=|
      | %<ID>
      | %<Vbase>V
      | %<VLF>pu
      | %<angleLF>deg.
      | %<Name>
  bus27 : powerlib/Measurements/Load Flow Bus  LConnTagsString=a  Phases=single  Connectors=on one side  ID=bus27  Vbase=220000  Vref=1  Vangle=0  VLF=1  VLFb=1  VLFc=1  angleLF=0  angleLFb=0  angleLFc=0
      settings: AttributesFormatString=|
      | %<ID>
      | %<Vbase>V
      | %<VLF>pu
      | %<angleLF>deg.
      | %<Name>
  bus28 : powerlib/Measurements/Load Flow Bus  LConnTagsString=a  Phases=single  Connectors=on one side  ID=bus28  Vbase=220000  Vref=1  Vangle=0  VLF=1  VLFb=1  VLFc=1  angleLF=0  angleLFb=0  angleLFc=0
      settings: AttributesFormatString=|
      | %<ID>
      | %<Vbase>V
      | %<VLF>pu
      | %<angleLF>deg.
      | %<Name>
  bus29 : powerlib/Measurements/Load Flow Bus  LConnTagsString=a  Phases=single  Connectors=on one side  ID=bus29  Vbase=220000  Vref=1  Vangle=0  VLF=1  VLFb=1  VLFc=1  angleLF=0  angleLFb=0  angleLFc=0
      settings: AttributesFormatString=|
      | %<ID>
      | %<Vbase>V
      | %<VLF>pu
      | %<angleLF>deg.
      | %<Name>
  bus3 : powerlib/Measurements/Load Flow Bus  LConnTagsString=a  Phases=single  Connectors=on one side  ID=bus3  Vbase=220000  Vref=1  Vangle=0  VLF=1  VLFb=1  VLFc=1  angleLF=0  angleLFb=0  angleLFc=0
      settings: AttributesFormatString=|
      | %<ID>
      | %<Vbase>V
      | %<VLF>pu
      | %<angleLF>deg.
      | %<Name>
  bus30 : powerlib/Measurements/Load Flow Bus  LConnTagsString=a  Phases=single  Connectors=on one side  ID=bus30  Vbase=220000  Vref=1  Vangle=0  VLF=1  VLFb=1  VLFc=1  angleLF=0  angleLFb=0  angleLFc=0
      settings: AttributesFormatString=|
      | %<ID>
      | %<Vbase>V
      | %<VLF>pu
      | %<angleLF>deg.
      | %<Name>
  bus31 : powerlib/Measurements/Load Flow Bus  LConnTagsString=a  Phases=single  Connectors=on one side  ID=bus31  Vbase=220000  Vref=1  Vangle=0  VLF=1  VLFb=1  VLFc=1  angleLF=0  angleLFb=0  angleLFc=0
      settings: AttributesFormatString=|
      | %<ID>
      | %<Vbase>V
      | %<VLF>pu
      | %<angleLF>deg.
      | %<Name>
  bus32 : powerlib/Measurements/Load Flow Bus  LConnTagsString=a  Phases=single  Connectors=on one side  ID=bus32  Vbase=220000  Vref=1  Vangle=0  VLF=1  VLFb=1  VLFc=1  angleLF=0  angleLFb=0  angleLFc=0
      settings: AttributesFormatString=|
      | %<ID>
      | %<Vbase>V
      | %<VLF>pu
      | %<angleLF>deg.
      | %<Name>
  bus33 : powerlib/Measurements/Load Flow Bus  LConnTagsString=a  Phases=single  Connectors=on one side  ID=bus33  Vbase=220000  Vref=1  Vangle=0  VLF=1  VLFb=1  VLFc=1  angleLF=0  angleLFb=0  angleLFc=0
      settings: AttributesFormatString=|
      | %<ID>
      | %<Vbase>V
      | %<VLF>pu
      | %<angleLF>deg.
      | %<Name>
  bus34 : powerlib/Measurements/Load Flow Bus  LConnTagsString=a  Phases=single  Connectors=on one side  ID=bus34  Vbase=220000  Vref=1  Vangle=0  VLF=1  VLFb=1  VLFc=1  angleLF=0  angleLFb=0  angleLFc=0
      settings: AttributesFormatString=|
      | %<ID>
      | %<Vbase>V
      | %<VLF>pu
      | %<angleLF>deg.
      | %<Name>
  bus35 : powerlib/Measurements/Load Flow Bus  LConnTagsString=a  Phases=single  Connectors=on one side  ID=bus35  Vbase=220000  Vref=1  Vangle=0  VLF=1  VLFb=1  VLFc=1  angleLF=0  angleLFb=0  angleLFc=0
      settings: AttributesFormatString=|
      | %<ID>
      | %<Vbase>V
      | %<VLF>pu
      | %<angleLF>deg.
      | %<Name>
  bus36 : powerlib/Measurements/Load Flow Bus  LConnTagsString=a  Phases=single  Connectors=on one side  ID=bus36  Vbase=220000  Vref=1  Vangle=0  VLF=1  VLFb=1  VLFc=1  angleLF=0  angleLFb=0  angleLFc=0
      settings: AttributesFormatString=|
      | %<ID>
      | %<Vbase>V
      | %<VLF>pu
      | %<angleLF>deg.
      | %<Name>
  bus37 : powerlib/Measurements/Load Flow Bus  LConnTagsString=a  Phases=single  Connectors=on one side  ID=bus37  Vbase=220000  Vref=1  Vangle=0  VLF=1  VLFb=1  VLFc=1  angleLF=0  angleLFb=0  angleLFc=0
      settings: AttributesFormatString=|
      | %<ID>
      | %<Vbase>V
      | %<VLF>pu
      | %<angleLF>deg.
      | %<Name>
  bus38 : powerlib/Measurements/Load Flow Bus  LConnTagsString=a  Phases=single  Connectors=on one side  ID=bus38  Vbase=220000  Vref=1  Vangle=0  VLF=1  VLFb=1  VLFc=1  angleLF=0  angleLFb=0  angleLFc=0
      settings: AttributesFormatString=|
      | %<ID>
      | %<Vbase>V
      | %<VLF>pu
      | %<angleLF>deg.
      | %<Name>
  bus39 : powerlib/Measurements/Load Flow Bus  LConnTagsString=a  Phases=single  Connectors=on one side  ID=bus39  Vbase=220000  Vref=1  Vangle=0  VLF=1  VLFb=1  VLFc=1  angleLF=0  angleLFb=0  angleLFc=0
      settings: AttributesFormatString=|
      | %<ID>
      | %<Vbase>V
      | %<VLF>pu
      | %<angleLF>deg.
      | %<Name>
  bus4 : powerlib/Measurements/Load Flow Bus  LConnTagsString=a  Phases=single  Connectors=on one side  ID=bus4  Vbase=220000  Vref=1  Vangle=0  VLF=1  VLFb=1  VLFc=1  angleLF=0  angleLFb=0  angleLFc=0
      settings: AttributesFormatString=|
      | %<ID>
      | %<Vbase>V
      | %<VLF>pu
      | %<angleLF>deg.
      | %<Name>
  bus40 : powerlib/Measurements/Load Flow Bus  LConnTagsString=a  Phases=single  Connectors=on one side  ID=bus40  Vbase=220000  Vref=1  Vangle=0  VLF=1  VLFb=1  VLFc=1  angleLF=0  angleLFb=0  angleLFc=0
      settings: AttributesFormatString=|
      | %<ID>
      | %<Vbase>V
      | %<VLF>pu
      | %<angleLF>deg.
      | %<Name>
  bus41 : powerlib/Measurements/Load Flow Bus  LConnTagsString=a  Phases=single  Connectors=on one side  ID=bus41  Vbase=220000  Vref=1  Vangle=0  VLF=1  VLFb=1  VLFc=1  angleLF=0  angleLFb=0  angleLFc=0
      settings: AttributesFormatString=|
      | %<ID>
      | %<Vbase>V
      | %<VLF>pu
      | %<angleLF>deg.
      | %<Name>
  bus42 : powerlib/Measurements/Load Flow Bus  LConnTagsString=a  Phases=single  Connectors=on one side  ID=bus42  Vbase=220000  Vref=1  Vangle=0  VLF=1  VLFb=1  VLFc=1  angleLF=0  angleLFb=0  angleLFc=0
      settings: AttributesFormatString=|
      | %<ID>
      | %<Vbase>V
      | %<VLF>pu
      | %<angleLF>deg.
      | %<Name>
  bus43 : powerlib/Measurements/Load Flow Bus  LConnTagsString=a  Phases=single  Connectors=on one side  ID=bus43  Vbase=220000  Vref=1  Vangle=0  VLF=1  VLFb=1  VLFc=1  angleLF=0  angleLFb=0  angleLFc=0
      settings: AttributesFormatString=|
      | %<ID>
      | %<Vbase>V
      | %<VLF>pu
      | %<angleLF>deg.
      | %<Name>
  bus44 : powerlib/Measurements/Load Flow Bus  LConnTagsString=a  Phases=single  Connectors=on one side  ID=bus44  Vbase=220000  Vref=1  Vangle=0  VLF=1  VLFb=1  VLFc=1  angleLF=0  angleLFb=0  angleLFc=0
      settings: AttributesFormatString=|
      | %<ID>
      | %<Vbase>V
      | %<VLF>pu
      | %<angleLF>deg.
      | %<Name>
  bus45 : powerlib/Measurements/Load Flow Bus  LConnTagsString=a  Phases=single  Connectors=on one side  ID=bus45  Vbase=220000  Vref=1  Vangle=0  VLF=1  VLFb=1  VLFc=1  angleLF=0  angleLFb=0  angleLFc=0
      settings: AttributesFormatString=|
      | %<ID>
      | %<Vbase>V
      | %<VLF>pu
      | %<angleLF>deg.
      | %<Name>
  bus46 : powerlib/Measurements/Load Flow Bus  LConnTagsString=a  Phases=single  Connectors=on one side  ID=bus46  Vbase=220000  Vref=1  Vangle=0  VLF=1  VLFb=1  VLFc=1  angleLF=0  angleLFb=0  angleLFc=0
      settings: AttributesFormatString=|
      | %<ID>
      | %<Vbase>V
      | %<VLF>pu
      | %<angleLF>deg.
      | %<Name>
  bus47 : powerlib/Measurements/Load Flow Bus  LConnTagsString=a  Phases=single  Connectors=on one side  ID=bus47  Vbase=220000  Vref=1  Vangle=0  VLF=1  VLFb=1  VLFc=1  angleLF=0  angleLFb=0  angleLFc=0
      settings: AttributesFormatString=|
      | %<ID>
      | %<Vbase>V
      | %<VLF>pu
      | %<angleLF>deg.
      | %<Name>
  bus48 : powerlib/Measurements/Load Flow Bus  LConnTagsString=a  Phases=single  Connectors=on one side  ID=bus48  Vbase=220000  Vref=1  Vangle=0  VLF=1  VLFb=1  VLFc=1  angleLF=0  angleLFb=0  angleLFc=0
      settings: AttributesFormatString=|
      | %<ID>
      | %<Vbase>V
      | %<VLF>pu
      | %<angleLF>deg.
      | %<Name>
  bus49 : powerlib/Measurements/Load Flow Bus  LConnTagsString=a  Phases=single  Connectors=on one side  ID=bus49  Vbase=220000  Vref=1  Vangle=0  VLF=1  VLFb=1  VLFc=1  angleLF=0  angleLFb=0  angleLFc=0
      settings: AttributesFormatString=|
      | %<ID>
      | %<Vbase>V
      | %<VLF>pu
      | %<angleLF>deg.
      | %<Name>
  bus5 : powerlib/Measurements/Load Flow Bus  LConnTagsString=a  Phases=single  Connectors=on one side  ID=bus5  Vbase=220000  Vref=1  Vangle=0  VLF=1  VLFb=1  VLFc=1  angleLF=0  angleLFb=0  angleLFc=0
      settings: AttributesFormatString=|
      | %<ID>
      | %<Vbase>V
      | %<VLF>pu
      | %<angleLF>deg.
      | %<Name>
  bus50 : powerlib/Measurements/Load Flow Bus  LConnTagsString=a  Phases=single  Connectors=on one side  ID=bus50  Vbase=220000  Vref=1  Vangle=0  VLF=1  VLFb=1  VLFc=1  angleLF=0  angleLFb=0  angleLFc=0
      settings: AttributesFormatString=|
      | %<ID>
      | %<Vbase>V
      | %<VLF>pu
      | %<angleLF>deg.
      | %<Name>
  bus51 : powerlib/Measurements/Load Flow Bus  LConnTagsString=a  Phases=single  Connectors=on one side  ID=bus51  Vbase=220000  Vref=1  Vangle=0  VLF=1  VLFb=1  VLFc=1  angleLF=0  angleLFb=0  angleLFc=0
      settings: AttributesFormatString=|
      | %<ID>
      | %<Vbase>V
      | %<VLF>pu
      | %<angleLF>deg.
      | %<Name>
  bus52 : powerlib/Measurements/Load Flow Bus  LConnTagsString=a  Phases=single  Connectors=on one side  ID=bus52  Vbase=220000  Vref=1  Vangle=0  VLF=1  VLFb=1  VLFc=1  angleLF=0  angleLFb=0  angleLFc=0
      settings: AttributesFormatString=|
      | %<ID>
      | %<Vbase>V
      | %<VLF>pu
      | %<angleLF>deg.
      | %<Name>
  bus53 : powerlib/Measurements/Load Flow Bus  LConnTagsString=a  Phases=single  Connectors=on one side  ID=bus53  Vbase=220000  Vref=1  Vangle=0  VLF=1  VLFb=1  VLFc=1  angleLF=0  angleLFb=0  angleLFc=0
      settings: AttributesFormatString=|
      | %<ID>
      | %<Vbase>V
      | %<VLF>pu
      | %<angleLF>deg.
      | %<Name>
  bus54 : powerlib/Measurements/Load Flow Bus  LConnTagsString=a  Phases=single  Connectors=on one side  ID=bus54  Vbase=220000  Vref=1  Vangle=0  VLF=1  VLFb=1  VLFc=1  angleLF=0  angleLFb=0  angleLFc=0
      settings: AttributesFormatString=|
      | %<ID>
      | %<Vbase>V
      | %<VLF>pu
      | %<angleLF>deg.
      | %<Name>
  bus55 : powerlib/Measurements/Load Flow Bus  LConnTagsString=a  Phases=single  Connectors=on one side  ID=bus55  Vbase=220000  Vref=1  Vangle=0  VLF=1  VLFb=1  VLFc=1  angleLF=0  angleLFb=0  angleLFc=0
      settings: AttributesFormatString=|
      | %<ID>
      | %<Vbase>V
      | %<VLF>pu
      | %<angleLF>deg.
      | %<Name>
  bus56 : powerlib/Measurements/Load Flow Bus  LConnTagsString=a  Phases=single  Connectors=on one side  ID=bus56  Vbase=220000  Vref=1  Vangle=0  VLF=1  VLFb=1  VLFc=1  angleLF=0  angleLFb=0  angleLFc=0
      settings: AttributesFormatString=|
      | %<ID>
      | %<Vbase>V
      | %<VLF>pu
      | %<angleLF>deg.
      | %<Name>
  bus57 : powerlib/Measurements/Load Flow Bus  LConnTagsString=a  Phases=single  Connectors=on one side  ID=bus57  Vbase=220000  Vref=1  Vangle=0  VLF=1  VLFb=1  VLFc=1  angleLF=0  angleLFb=0  angleLFc=0
      settings: AttributesFormatString=|
      | %<ID>
      | %<Vbase>V
      | %<VLF>pu
      | %<angleLF>deg.
      | %<Name>
  bus58 : powerlib/Measurements/Load Flow Bus  LConnTagsString=a  Phases=single  Connectors=on one side  ID=bus58  Vbase=220000  Vref=1  Vangle=0  VLF=1  VLFb=1  VLFc=1  angleLF=0  angleLFb=0  angleLFc=0
      settings: AttributesFormatString=|
      | %<ID>
      | %<Vbase>V
      | %<VLF>pu
      | %<angleLF>deg.
      | %<Name>
  bus59 : powerlib/Measurements/Load Flow Bus  LConnTagsString=a  Phases=single  Connectors=on one side  ID=bus59  Vbase=220000  Vref=1  Vangle=0  VLF=1  VLFb=1  VLFc=1  angleLF=0  angleLFb=0  angleLFc=0
      settings: AttributesFormatString=|
      | %<ID>
      | %<Vbase>V
      | %<VLF>pu
      | %<angleLF>deg.
      | %<Name>
  bus6 : powerlib/Measurements/Load Flow Bus  LConnTagsString=a  Phases=single  Connectors=on one side  ID=bus6  Vbase=220000  Vref=1  Vangle=0  VLF=1  VLFb=1  VLFc=1  angleLF=0  angleLFb=0  angleLFc=0
      settings: AttributesFormatString=|
      | %<ID>
      | %<Vbase>V
      | %<VLF>pu
      | %<angleLF>deg.
      | %<Name>
  bus60 : powerlib/Measurements/Load Flow Bus  LConnTagsString=a  Phases=single  Connectors=on one side  ID=bus60  Vbase=220000  Vref=1  Vangle=0  VLF=1  VLFb=1  VLFc=1  angleLF=0  angleLFb=0  angleLFc=0
      settings: AttributesFormatString=|
      | %<ID>
      | %<Vbase>V
      | %<VLF>pu
      | %<angleLF>deg.
      | %<Name>
  bus61 : powerlib/Measurements/Load Flow Bus  LConnTagsString=a  Phases=single  Connectors=on one side  ID=bus61  Vbase=220000  Vref=1  Vangle=0  VLF=1  VLFb=1  VLFc=1  angleLF=0  angleLFb=0  angleLFc=0
      settings: AttributesFormatString=|
      | %<ID>
      | %<Vbase>V
      | %<VLF>pu
      | %<angleLF>deg.
      | %<Name>
  bus62 : powerlib/Measurements/Load Flow Bus  LConnTagsString=a  Phases=single  Connectors=on one side  ID=bus62  Vbase=220000  Vref=1  Vangle=0  VLF=1  VLFb=1  VLFc=1  angleLF=0  angleLFb=0  angleLFc=0
      settings: AttributesFormatString=|
      | %<ID>
      | %<Vbase>V
      | %<VLF>pu
      | %<angleLF>deg.
      | %<Name>
  bus63 : powerlib/Measurements/Load Flow Bus  LConnTagsString=a  Phases=single  Connectors=on one side  ID=bus63  Vbase=220000  Vref=1  Vangle=0  VLF=1  VLFb=1  VLFc=1  angleLF=0  angleLFb=0  angleLFc=0
      settings: AttributesFormatString=|
      | %<ID>
      | %<Vbase>V
      | %<VLF>pu
      | %<angleLF>deg.
      | %<Name>
  bus64 : powerlib/Measurements/Load Flow Bus  LConnTagsString=a  Phases=single  Connectors=on one side  ID=bus64  Vbase=220000  Vref=1  Vangle=0  VLF=1  VLFb=1  VLFc=1  angleLF=0  angleLFb=0  angleLFc=0
      settings: AttributesFormatString=|
      | %<ID>
      | %<Vbase>V
      | %<VLF>pu
      | %<angleLF>deg.
      | %<Name>
  bus65 : powerlib/Measurements/Load Flow Bus  LConnTagsString=a  Phases=single  Connectors=on one side  ID=bus65  Vbase=220000  Vref=1  Vangle=0  VLF=1  VLFb=1  VLFc=1  angleLF=0  angleLFb=0  angleLFc=0
      settings: AttributesFormatString=|
      | %<ID>
      | %<Vbase>V
      | %<VLF>pu
      | %<angleLF>deg.
      | %<Name>
  bus66 : powerlib/Measurements/Load Flow Bus  LConnTagsString=a  Phases=single  Connectors=on one side  ID=bus66  Vbase=220000  Vref=1  Vangle=0  VLF=1  VLFb=1  VLFc=1  angleLF=0  angleLFb=0  angleLFc=0
      settings: AttributesFormatString=|
      | %<ID>
      | %<Vbase>V
      | %<VLF>pu
      | %<angleLF>deg.
      | %<Name>
  bus67 : powerlib/Measurements/Load Flow Bus  LConnTagsString=a  Phases=single  Connectors=on one side  ID=bus67  Vbase=220000  Vref=1  Vangle=0  VLF=1  VLFb=1  VLFc=1  angleLF=0  angleLFb=0  angleLFc=0
      settings: AttributesFormatString=|
      | %<ID>
      | %<Vbase>V
      | %<VLF>pu
      | %<angleLF>deg.
      | %<Name>
  bus68 : powerlib/Measurements/Load Flow Bus  LConnTagsString=a  Phases=single  Connectors=on one side  ID=bus68  Vbase=220000  Vref=1  Vangle=0  VLF=1  VLFb=1  VLFc=1  angleLF=0  angleLFb=0  angleLFc=0
      settings: AttributesFormatString=|
      | %<ID>
      | %<Vbase>V
      | %<VLF>pu
      | %<angleLF>deg.
      | %<Name>
  bus69 : powerlib/Measurements/Load Flow Bus  LConnTagsString=a  Phases=single  Connectors=on one side  ID=bus69  Vbase=220000  Vref=1  Vangle=0  VLF=1  VLFb=1  VLFc=1  angleLF=0  angleLFb=0  angleLFc=0
      settings: AttributesFormatString=|
      | %<ID>
      | %<Vbase>V
      | %<VLF>pu
      | %<angleLF>deg.
      | %<Name>
  bus7 : powerlib/Measurements/Load Flow Bus  LConnTagsString=a  Phases=single  Connectors=on one side  ID=bus7  Vbase=220000  Vref=1  Vangle=0  VLF=1  VLFb=1  VLFc=1  angleLF=0  angleLFb=0  angleLFc=0
      settings: AttributesFormatString=|
      | %<ID>
      | %<Vbase>V
      | %<VLF>pu
      | %<angleLF>deg.
      | %<Name>
  bus70 : powerlib/Measurements/Load Flow Bus  LConnTagsString=a  Phases=single  Connectors=on one side  ID=bus70  Vbase=220000  Vref=1  Vangle=0  VLF=1  VLFb=1  VLFc=1  angleLF=0  angleLFb=0  angleLFc=0
      settings: AttributesFormatString=|
      | %<ID>
      | %<Vbase>V
      | %<VLF>pu
      | %<angleLF>deg.
      | %<Name>
  bus71 : powerlib/Measurements/Load Flow Bus  LConnTagsString=a  Phases=single  Connectors=on one side  ID=bus71  Vbase=220000  Vref=1  Vangle=0  VLF=1  VLFb=1  VLFc=1  angleLF=0  angleLFb=0  angleLFc=0
      settings: AttributesFormatString=|
      | %<ID>
      | %<Vbase>V
      | %<VLF>pu
      | %<angleLF>deg.
      | %<Name>
  bus72 : powerlib/Measurements/Load Flow Bus  LConnTagsString=a  Phases=single  Connectors=on one side  ID=bus72  Vbase=220000  Vref=1  Vangle=0  VLF=1  VLFb=1  VLFc=1  angleLF=0  angleLFb=0  angleLFc=0
      settings: AttributesFormatString=|
      | %<ID>
      | %<Vbase>V
      | %<VLF>pu
      | %<angleLF>deg.
      | %<Name>
  bus73 : powerlib/Measurements/Load Flow Bus  LConnTagsString=a  Phases=single  Connectors=on one side  ID=bus73  Vbase=220000  Vref=1  Vangle=0  VLF=1  VLFb=1  VLFc=1  angleLF=0  angleLFb=0  angleLFc=0
      settings: AttributesFormatString=|
      | %<ID>
      | %<Vbase>V
      | %<VLF>pu
      | %<angleLF>deg.
      | %<Name>
  bus74 : powerlib/Measurements/Load Flow Bus  LConnTagsString=a  Phases=single  Connectors=on one side  ID=bus74  Vbase=220000  Vref=1  Vangle=0  VLF=1  VLFb=1  VLFc=1  angleLF=0  angleLFb=0  angleLFc=0
      settings: AttributesFormatString=|
      | %<ID>
      | %<Vbase>V
      | %<VLF>pu
      | %<angleLF>deg.
      | %<Name>
  bus75 : powerlib/Measurements/Load Flow Bus  LConnTagsString=a  Phases=single  Connectors=on one side  ID=bus75  Vbase=220000  Vref=1  Vangle=0  VLF=1  VLFb=1  VLFc=1  angleLF=0  angleLFb=0  angleLFc=0
      settings: AttributesFormatString=|
      | %<ID>
      | %<Vbase>V
      | %<VLF>pu
      | %<angleLF>deg.
      | %<Name>
  bus76 : powerlib/Measurements/Load Flow Bus  LConnTagsString=a  Phases=single  Connectors=on one side  ID=bus76  Vbase=220000  Vref=1  Vangle=0  VLF=1  VLFb=1  VLFc=1  angleLF=0  angleLFb=0  angleLFc=0
      settings: AttributesFormatString=|
      | %<ID>
      | %<Vbase>V
      | %<VLF>pu
      | %<angleLF>deg.
      | %<Name>
  bus77 : powerlib/Measurements/Load Flow Bus  LConnTagsString=a  Phases=single  Connectors=on one side  ID=bus77  Vbase=220000  Vref=1  Vangle=0  VLF=1  VLFb=1  VLFc=1  angleLF=0  angleLFb=0  angleLFc=0
      settings: AttributesFormatString=|
      | %<ID>
      | %<Vbase>V
      | %<VLF>pu
      | %<angleLF>deg.
      | %<Name>
  bus78 : powerlib/Measurements/Load Flow Bus  LConnTagsString=a  Phases=single  Connectors=on one side  ID=bus78  Vbase=220000  Vref=1  Vangle=0  VLF=1  VLFb=1  VLFc=1  angleLF=0  angleLFb=0  angleLFc=0
      settings: AttributesFormatString=|
      | %<ID>
      | %<Vbase>V
      | %<VLF>pu
      | %<angleLF>deg.
      | %<Name>
  bus79 : powerlib/Measurements/Load Flow Bus  LConnTagsString=a  Phases=single  Connectors=on one side  ID=bus79  Vbase=220000  Vref=1  Vangle=0  VLF=1  VLFb=1  VLFc=1  angleLF=0  angleLFb=0  angleLFc=0
      settings: AttributesFormatString=|
      | %<ID>
      | %<Vbase>V
      | %<VLF>pu
      | %<angleLF>deg.
      | %<Name>
  bus8 : powerlib/Measurements/Load Flow Bus  LConnTagsString=a  Phases=single  Connectors=on one side  ID=bus8  Vbase=220000  Vref=1  Vangle=0  VLF=1  VLFb=1  VLFc=1  angleLF=0  angleLFb=0  angleLFc=0
      settings: AttributesFormatString=|
      | %<ID>
      | %<Vbase>V
      | %<VLF>pu
      | %<angleLF>deg.
      | %<Name>
  bus80 : powerlib/Measurements/Load Flow Bus  LConnTagsString=a  Phases=single  Connectors=on one side  ID=bus80  Vbase=220000  Vref=1  Vangle=0  VLF=1  VLFb=1  VLFc=1  angleLF=0  angleLFb=0  angleLFc=0
      settings: AttributesFormatString=|
      | %<ID>
      | %<Vbase>V
      | %<VLF>pu
      | %<angleLF>deg.
      | %<Name>
  bus81 : powerlib/Measurements/Load Flow Bus  LConnTagsString=a  Phases=single  Connectors=on one side  ID=bus81  Vbase=220000  Vref=1  Vangle=0  VLF=1  VLFb=1  VLFc=1  angleLF=0  angleLFb=0  angleLFc=0
      settings: AttributesFormatString=|
      | %<ID>
      | %<Vbase>V
      | %<VLF>pu
      | %<angleLF>deg.
      | %<Name>
  bus82 : powerlib/Measurements/Load Flow Bus  LConnTagsString=a  Phases=single  Connectors=on one side  ID=bus82  Vbase=220000  Vref=1  Vangle=0  VLF=1  VLFb=1  VLFc=1  angleLF=0  angleLFb=0  angleLFc=0
      settings: AttributesFormatString=|
      | %<ID>
      | %<Vbase>V
      | %<VLF>pu
      | %<angleLF>deg.
      | %<Name>
  bus83 : powerlib/Measurements/Load Flow Bus  LConnTagsString=a  Phases=single  Connectors=on one side  ID=bus83  Vbase=220000  Vref=1  Vangle=0  VLF=1  VLFb=1  VLFc=1  angleLF=0  angleLFb=0  angleLFc=0
      settings: AttributesFormatString=|
      | %<ID>
      | %<Vbase>V
      | %<VLF>pu
      | %<angleLF>deg.
      | %<Name>
  bus84 : powerlib/Measurements/Load Flow Bus  LConnTagsString=a  Phases=single  Connectors=on one side  ID=bus84  Vbase=220000  Vref=1  Vangle=0  VLF=1  VLFb=1  VLFc=1  angleLF=0  angleLFb=0  angleLFc=0
      settings: AttributesFormatString=|
      | %<ID>
      | %<Vbase>V
      | %<VLF>pu
      | %<angleLF>deg.
      | %<Name>
  bus85 : powerlib/Measurements/Load Flow Bus  LConnTagsString=a  Phases=single  Connectors=on one side  ID=bus85  Vbase=220000  Vref=1  Vangle=0  VLF=1  VLFb=1  VLFc=1  angleLF=0  angleLFb=0  angleLFc=0
      settings: AttributesFormatString=|
      | %<ID>
      | %<Vbase>V
      | %<VLF>pu
      | %<angleLF>deg.
      | %<Name>
  bus86 : powerlib/Measurements/Load Flow Bus  LConnTagsString=a  Phases=single  Connectors=on one side  ID=bus86  Vbase=220000  Vref=1  Vangle=0  VLF=1  VLFb=1  VLFc=1  angleLF=0  angleLFb=0  angleLFc=0
      settings: AttributesFormatString=|
      | %<ID>
      | %<Vbase>V
      | %<VLF>pu
      | %<angleLF>deg.
      | %<Name>
  bus87 : powerlib/Measurements/Load Flow Bus  LConnTagsString=a  Phases=single  Connectors=on one side  ID=bus87  Vbase=220000  Vref=1  Vangle=0  VLF=1  VLFb=1  VLFc=1  angleLF=0  angleLFb=0  angleLFc=0
      settings: AttributesFormatString=|
      | %<ID>
      | %<Vbase>V
      | %<VLF>pu
      | %<angleLF>deg.
      | %<Name>
  bus88 : powerlib/Measurements/Load Flow Bus  LConnTagsString=a  Phases=single  Connectors=on one side  ID=bus88  Vbase=220000  Vref=1  Vangle=0  VLF=1  VLFb=1  VLFc=1  angleLF=0  angleLFb=0  angleLFc=0
      settings: AttributesFormatString=|
      | %<ID>
      | %<Vbase>V
      | %<VLF>pu
      | %<angleLF>deg.
      | %<Name>
  bus89 : powerlib/Measurements/Load Flow Bus  LConnTagsString=a  Phases=single  Connectors=on one side  ID=bus89  Vbase=220000  Vref=1  Vangle=0  VLF=1  VLFb=1  VLFc=1  angleLF=0  angleLFb=0  angleLFc=0
      settings: AttributesFormatString=|
      | %<ID>
      | %<Vbase>V
      | %<VLF>pu
      | %<angleLF>deg.
      | %<Name>
  bus9 : powerlib/Measurements/Load Flow Bus  LConnTagsString=a  Phases=single  Connectors=on one side  ID=bus9  Vbase=220000  Vref=1  Vangle=0  VLF=1  VLFb=1  VLFc=1  angleLF=0  angleLFb=0  angleLFc=0
      settings: AttributesFormatString=|
      | %<ID>
      | %<Vbase>V
      | %<VLF>pu
      | %<angleLF>deg.
      | %<Name>
  bus90 : powerlib/Measurements/Load Flow Bus  LConnTagsString=a  Phases=single  Connectors=on one side  ID=bus90  Vbase=220000  Vref=1  Vangle=0  VLF=1  VLFb=1  VLFc=1  angleLF=0  angleLFb=0  angleLFc=0
      settings: AttributesFormatString=|
      | %<ID>
      | %<Vbase>V
      | %<VLF>pu
      | %<angleLF>deg.
      | %<Name>
  bus91 : powerlib/Measurements/Load Flow Bus  LConnTagsString=a  Phases=single  Connectors=on one side  ID=bus91  Vbase=220000  Vref=1  Vangle=0  VLF=1  VLFb=1  VLFc=1  angleLF=0  angleLFb=0  angleLFc=0
      settings: AttributesFormatString=|
      | %<ID>
      | %<Vbase>V
      | %<VLF>pu
      | %<angleLF>deg.
      | %<Name>
  bus92 : powerlib/Measurements/Load Flow Bus  LConnTagsString=a  Phases=single  Connectors=on one side  ID=bus92  Vbase=220000  Vref=1  Vangle=0  VLF=1  VLFb=1  VLFc=1  angleLF=0  angleLFb=0  angleLFc=0
      settings: AttributesFormatString=|
      | %<ID>
      | %<Vbase>V
      | %<VLF>pu
      | %<angleLF>deg.
      | %<Name>
  bus93 : powerlib/Measurements/Load Flow Bus  LConnTagsString=a  Phases=single  Connectors=on one side  ID=bus93  Vbase=220000  Vref=1  Vangle=0  VLF=1  VLFb=1  VLFc=1  angleLF=0  angleLFb=0  angleLFc=0
      settings: AttributesFormatString=|
      | %<ID>
      | %<Vbase>V
      | %<VLF>pu
      | %<angleLF>deg.
      | %<Name>
  bus94 : powerlib/Measurements/Load Flow Bus  LConnTagsString=a  Phases=single  Connectors=on one side  ID=bus94  Vbase=220000  Vref=1  Vangle=0  VLF=1  VLFb=1  VLFc=1  angleLF=0  angleLFb=0  angleLFc=0
      settings: AttributesFormatString=|
      | %<ID>
      | %<Vbase>V
      | %<VLF>pu
      | %<angleLF>deg.
      | %<Name>
  bus95 : powerlib/Measurements/Load Flow Bus  LConnTagsString=a  Phases=single  Connectors=on one side  ID=bus95  Vbase=220000  Vref=1  Vangle=0  VLF=1  VLFb=1  VLFc=1  angleLF=0  angleLFb=0  angleLFc=0
      settings: AttributesFormatString=|
      | %<ID>
      | %<Vbase>V
      | %<VLF>pu
      | %<angleLF>deg.
      | %<Name>
  bus96 : powerlib/Measurements/Load Flow Bus  LConnTagsString=a  Phases=single  Connectors=on one side  ID=bus96  Vbase=220000  Vref=1  Vangle=0  VLF=1  VLFb=1  VLFc=1  angleLF=0  angleLFb=0  angleLFc=0
      settings: AttributesFormatString=|
      | %<ID>
      | %<Vbase>V
      | %<VLF>pu
      | %<angleLF>deg.
      | %<Name>
  bus97 : powerlib/Measurements/Load Flow Bus  LConnTagsString=a  Phases=single  Connectors=on one side  ID=bus97  Vbase=220000  Vref=1  Vangle=0  VLF=1  VLFb=1  VLFc=1  angleLF=0  angleLFb=0  angleLFc=0
      settings: AttributesFormatString=|
      | %<ID>
      | %<Vbase>V
      | %<VLF>pu
      | %<angleLF>deg.
      | %<Name>
  bus98 : powerlib/Measurements/Load Flow Bus  LConnTagsString=a  Phases=single  Connectors=on one side  ID=bus98  Vbase=220000  Vref=1  Vangle=0  VLF=1  VLFb=1  VLFc=1  angleLF=0  angleLFb=0  angleLFc=0
      settings: AttributesFormatString=|
      | %<ID>
      | %<Vbase>V
      | %<VLF>pu
      | %<angleLF>deg.
      | %<Name>
  bus99 : powerlib/Measurements/Load Flow Bus  LConnTagsString=a  Phases=single  Connectors=on one side  ID=bus99  Vbase=220000  Vref=1  Vangle=0  VLF=1  VLFb=1  VLFc=1  angleLF=0  angleLFb=0  angleLFc=0
      settings: AttributesFormatString=|
      | %<ID>
      | %<Vbase>V
      | %<VLF>pu
      | %<angleLF>deg.
      | %<Name>
  powergui : powerlib/powergui  Priority=1  SimulationMode=Phasor  SolverType=Tustin/Backward Euler (TBE)  SampleTime=50e-6  frequency=50  SPID=off  DisableSnubberDevices=off  DisableRonSwitches=off  DisableVfSwitches=off  SwTol=0  DisplayEquations=off  Interpol=off  ExternalGateDelay=off  methode=off  Ts=10  FunctionMessages=off  echomessages=off  HookPort=off  EnableUseOfTLC=off  x0status=blocks  frequencyindice=50  Pbase=3000e6  ErrMax=0.0001  Iterations=50  UnitsV=V  UnitsW=W  buscounter=0  RestoreLinks=warning  ResistiveCurrentMeasurement=off  Frange=[0:2:500]  Ylog=off  Xlog=on  ShowGrid=off  save=off  variable=ZData  structure=0  ZoomFFT=off  StartTime=0.0  cycles=1  DisplayStyle=1  fundamental=60  FreqAxis=off  MaxFrequency=1000  frequencyindicesteady=1  RmsSteady=1  display=off
  system_1_CN_305265212_400000_CN_365677253_400000 : powerlib/Elements/Distributed Parameters Line  Phases=3  Frequency=50  Resistance=[0.01273 0.3864]  Inductance="[0.9337e-3  4.1264e-3]"  Capacitance=[12.74e-9 7.751e-9]  Length=0.052476  x1=[8.73114913702011e-11 380000 380000;314.159265358979 314.159265358979 314.159265358979;-0.177670123217348 0.415246442777429 -1.15554988401747]  x2=[1.26090477118469e-09 381852.398472139 381852.398472139;314.159265358979 314.159265358979 314.159265358979;-1.41941675517191 0.415007521738739 -1.15578880505616]  x3=[1.07663708898761e-11 1405.24743813465 1405.24743813466;314.159265358979 314.159265358979 314.159265358979;-2.70558821102223 0.316110507002444 -1.25468581979246]  x4=[8.62234243168895e-12 1405.96374414071 1405.9637441407;314.159265358979 314.159265358979 314.159265358979;0.245769282942371 0.405640215255436 -1.16515611153945]  x5=0.000565541566995742  V1=ones(3,3)  V2=ones(3,3)  I1=ones(3,3)  I2=ones(3,3)  nHarmo=1  Measurements=None
  Świebodzice___Wrocław_CN_276291999_400000_CN_154510504_400000 : powerlib/Elements/Distributed Parameters Line  Phases=3  Frequency=50  Resistance=[0.01273 0.3864]  Inductance="[0.9337e-3  4.1264e-3]"  Capacitance=[12.74e-9 7.751e-9]  Length=43.0412  x1=[8.73114913702011e-11 380000 380000;314.159265358979 314.159265358979 314.159265358979;-0.177670123217348 0.415246442777429 -1.15554988401747]  x2=[1.26090477118469e-09 381852.398472139 381852.398472139;314.159265358979 314.159265358979 314.159265358979;-1.41941675517191 0.415007521738739 -1.15578880505616]  x3=[1.07663708898761e-11 1405.24743813465 1405.24743813466;314.159265358979 314.159265358979 314.159265358979;-2.70558821102223 0.316110507002444 -1.25468581979246]  x4=[8.62234243168895e-12 1405.96374414071 1405.9637441407;314.159265358979 314.159265358979 314.159265358979;0.245769282942371 0.405640215255436 -1.16515611153945]  x5=0.000565541566995742  V1=ones(3,3)  V2=ones(3,3)  I1=ones(3,3)  I2=ones(3,3)  nHarmo=1  Measurements=None
  connections:
  220kV_Lubocza___Wanda_CN_87667718_220000_CN_191035265_220000/LConn1 -- "T_87667718_220000;110000_Stacja_elektroenergetyczna_\"Lubocza\"_220_110kV"/LConn1 -- 220kV_Siersza___Lubocza_CN_87667718_220000_CN_187420591_220000/LConn1 -- 220kV_Lubocza___Wanda_CN_87667718_220000_CN_179864449_220000/LConn1 -- 220kV_Lubocza___Wanda_CN_87667718_220000_CN_115801644_220000/LConn1
  220kV_Lubocza___Wanda_CN_87667718_220000_CN_191035265_220000/LConn2 -- "T_87667718_220000;110000_Stacja_elektroenergetyczna_\"Lubocza\"_220_110kV"/LConn2 -- 220kV_Siersza___Lubocza_CN_87667718_220000_CN_187420591_220000/LConn2 -- 220kV_Lubocza___Wanda_CN_87667718_220000_CN_179864449_220000/LConn2 -- 220kV_Lubocza___Wanda_CN_87667718_220000_CN_115801644_220000/LConn2
  220kV_Lubocza___Wanda_CN_87667718_220000_CN_191035265_220000/LConn3 -- "T_87667718_220000;110000_Stacja_elektroenergetyczna_\"Lubocza\"_220_110kV"/LConn3 -- 220kV_Siersza___Lubocza_CN_87667718_220000_CN_187420591_220000/LConn3 -- bus1/LConn1 -- 220kV_Lubocza___Wanda_CN_87667718_220000_CN_179864449_220000/LConn3 -- 220kV_Lubocza___Wanda_CN_87667718_220000_CN_115801644_220000/LConn3
  220kV_Lubocza___Wanda_CN_87667718_220000_CN_191035265_220000/RConn1 -- "T_191035265_220000;110000_Stacja_elektroenergetyczna_\"Klikowa\"_220_110_kV"/LConn1 -- 220kV_Klikowa___Azoty_Tarnów_CN_191038569_220000_CN_191035265_220000/LConn1
  220kV_Lubocza___Wanda_CN_87667718_220000_CN_191035265_220000/RConn2 -- "T_191035265_220000;110000_Stacja_elektroenergetyczna_\"Klikowa\"_220_110_kV"/LConn2 -- 220kV_Klikowa___Azoty_Tarnów_CN_191038569_220000_CN_191035265_220000/LConn2
  220kV_Lubocza___Wanda_CN_87667718_220000_CN_191035265_220000/RConn3 -- "T_191035265_220000;110000_Stacja_elektroenergetyczna_\"Klikowa\"_220_110_kV"/LConn3 -- 220kV_Klikowa___Azoty_Tarnów_CN_191038569_220000_CN_191035265_220000/LConn3 -- bus2/LConn1
  220kV_Lubocza___Wanda_CN_87667718_220000_CN_179864449_220000/RConn1 -- G_179864449_Elektrownia_Skawina_S_A_/RConn1 -- 220kV_Byczyna___Skawina_CN_133537926_220000_CN_179864449_220000/LConn1
  220kV_Lubocza___Wanda_CN_87667718_220000_CN_179864449_220000/RConn2 -- G_179864449_Elektrownia_Skawina_S_A_/RConn2 -- 220kV_Byczyna___Skawina_CN_133537926_220000_CN_179864449_220000/LConn2
  220kV_Lubocza___Wanda_CN_87667718_220000_CN_179864449_220000/RConn3 -- G_179864449_Elektrownia_Skawina_S_A_/RConn3 -- 220kV_Byczyna___Skawina_CN_133537926_220000_CN_179864449_220000/LConn3 -- bus3/LConn1
  T_115801644_220000;110000_Stacja_elektroenergetyczna_„Wanda”_220_110_kV/LConn1 -- 220kV_Lubocza___Wanda_CN_87667718_220000_CN_115801644_220000/RConn1
  T_115801644_220000;110000_Stacja_elektroenergetyczna_„Wanda”_220_110_kV/LConn2 -- 220kV_Lubocza___Wanda_CN_87667718_220000_CN_115801644_220000/RConn2
  220kV_Lubocza___Wanda_CN_87667718_220000_CN_115801644_220000/RConn3 -- T_115801644_220000;110000_Stacja_elektroenergetyczna_„Wanda”_220_110_kV/LConn3 -- bus4/LConn1
  220kV_Siersza___Lubocza_CN_87667718_220000_CN_187420591_220000/RConn1 -- T_187420591_220000;110000_Stacja_elektroenergetyczna_„Siersza”_220_110kV/LConn1 -- 220kV_Byczyna___Skawina_CN_133537926_220000_CN_187420591_220000/LConn1 -- 220kV_Koksochemia___Łośnice_CN_66051759_220000_CN_187420591_220000/LConn1
  220kV_Siersza___Lubocza_CN_87667718_220000_CN_187420591_220000/RConn2 -- T_187420591_220000;110000_Stacja_elektroenergetyczna_„Siersza”_220_110kV/LConn2 -- 220kV_Byczyna___Skawina_CN_133537926_220000_CN_187420591_220000/LConn2 -- 220kV_Koksochemia___Łośnice_CN_66051759_220000_CN_187420591_220000/LConn2
  220kV_Siersza___Lubocza_CN_87667718_220000_CN_187420591_220000/RConn3 -- T_187420591_220000;110000_Stacja_elektroenergetyczna_„Siersza”_220_110kV/LConn3 -- 220kV_Byczyna___Skawina_CN_133537926_220000_CN_187420591_220000/LConn3 -- 220kV_Koksochemia___Łośnice_CN_66051759_220000_CN_187420591_220000/LConn3 -- bus5/LConn1
  220kV_Krajnik___Gorzów_CN_223873553_220000_CN_39428977_220000/LConn1 -- "T_223873553_220000;110000_Stacja_elektroenergetyczna_\"Gorzów\"_220_110_kV"/LConn1 -- 220kV_Leśniów___Gorzów_CN_223873553_220000_CN_158232924_220000/LConn1
  220kV_Krajnik___Gorzów_CN_223873553_220000_CN_39428977_220000/LConn2 -- "T_223873553_220000;110000_Stacja_elektroenergetyczna_\"Gorzów\"_220_110_kV"/LConn2 -- 220kV_Leśniów___Gorzów_CN_223873553_220000_CN_158232924_220000/LConn2
  220kV_Krajnik___Gorzów_CN_223873553_220000_CN_39428977_220000/LConn3 -- "T_223873553_220000;110000_Stacja_elektroenergetyczna_\"Gorzów\"_220_110_kV"/LConn3 -- 220kV_Leśniów___Gorzów_CN_223873553_220000_CN_158232924_220000/LConn3 -- bus6/LConn1
  220kV_Krajnik___Gorzów_CN_223873553_220000_CN_39428977_220000/RConn1 -- "T_39428977_400000;220000_Stacja_elektroenergetyczna_\"Krajnik\"_400_220_kV"/RConn1 -- _CN_39428977_220000_CN_35222596_220000/LConn1 -- _CN_39428977_220000_CN_177493901_220000/LConn1 -- 220kV_Krajnik___Glinki_CN_39428977_220000_CN_40062974_220000/LConn1 -- L_39428977/LConn1 -- 220kV_Krajnik___Morzyczyn_CN_32943179_220000_CN_39428977_220000/LConn1
  220kV_Krajnik___Gorzów_CN_223873553_220000_CN_39428977_220000/RConn2 -- "T_39428977_400000;220000_Stacja_elektroenergetyczna_\"Krajnik\"_400_220_kV"/RConn2 -- _CN_39428977_220000_CN_35222596_220000/LConn2 -- _CN_39428977_220000_CN_177493901_220000/LConn2 -- 220kV_Krajnik___Glinki_CN_39428977_220000_CN_40062974_220000/LConn2 -- L_39428977/LConn2 -- 220kV_Krajnik___Morzyczyn_CN_32943179_220000_CN_39428977_220000/LConn2
  220kV_Krajnik___Gorzów_CN_223873553_220000_CN_39428977_220000/RConn3 -- "T_39428977_400000;220000_Stacja_elektroenergetyczna_\"Krajnik\"_400_220_kV"/RConn3 -- _CN_39428977_220000_CN_35222596_220000/LConn3 -- _CN_39428977_220000_CN_177493901_220000/LConn3 -- 220kV_Krajnik___Glinki_CN_39428977_220000_CN_40062974_220000/LConn3 -- L_39428977/LConn3 -- bus7/LConn1 -- 220kV_Krajnik___Morzyczyn_CN_32943179_220000_CN_39428977_220000/LConn3
  220kV_Leśniów___Gorzów_CN_223873553_220000_CN_158232924_220000/RConn1 -- "T_158232924_220000;110000_Stacja_elektroenergetyczna_\"Leśniów\"_220_110_kV"/LConn1 -- 220kV_Leśniów___Zielona_Góra_CN_158232924_220000_CN_221120858_220000/LConn1 -- 220kV_Leśniów___Żukowice_CN_180535363_220000_CN_158232924_220000/LConn1 -- 220kV_Mikułowa___Leśniów_CN_111615226_220000_CN_158232924_220000/LConn1
  220kV_Leśniów___Gorzów_CN_223873553_220000_CN_158232924_220000/RConn2 -- "T_158232924_220000;110000_Stacja_elektroenergetyczna_\"Leśniów\"_220_110_kV"/LConn2 -- 220kV_Leśniów___Zielona_Góra_CN_158232924_220000_CN_221120858_220000/LConn2 -- 220kV_Leśniów___Żukowice_CN_180535363_220000_CN_158232924_220000/LConn2 -- 220kV_Mikułowa___Leśniów_CN_111615226_220000_CN_158232924_220000/LConn2
  220kV_Leśniów___Gorzów_CN_223873553_220000_CN_158232924_220000/RConn3 -- "T_158232924_220000;110000_Stacja_elektroenergetyczna_\"Leśniów\"_220_110_kV"/LConn3 -- 220kV_Leśniów___Zielona_Góra_CN_158232924_220000_CN_221120858_220000/LConn3 -- bus8/LConn1 -- 220kV_Leśniów___Żukowice_CN_180535363_220000_CN_158232924_220000/LConn3 -- 220kV_Mikułowa___Leśniów_CN_111615226_220000_CN_158232924_220000/LConn3
  220kV_Konin___Adamów_I_CN_171383831_220000_CN_216975352_220000/LConn1 -- T_171383831_220000;110000_Stacja_elektroenergetyczna_Adamów_220_110_kV/LConn1 -- 220kV_Adamów___Zgierz_CN_171383831_220000_CN_35366436_220000/LConn1 -- 220kV_Adamów___Zgierz_CN_171383831_220000_CN_101982559_220000/LConn1 -- 220kV_Adamów___Pabianice_CN_171383831_220000_CN_102165724_220000/LConn1 -- _CN_171383831_220000_CN_171385683_220000/LConn1
  220kV_Konin___Adamów_I_CN_171383831_220000_CN_216975352_220000/LConn2 -- T_171383831_220000;110000_Stacja_elektroenergetyczna_Adamów_220_110_kV/LConn2 -- 220kV_Adamów___Zgierz_CN_171383831_220000_CN_35366436_220000/LConn2 -- 220kV_Adamów___Zgierz_CN_171383831_220000_CN_101982559_220000/LConn2 -- 220kV_Adamów___Pabianice_CN_171383831_220000_CN_102165724_220000/LConn2 -- _CN_171383831_220000_CN_171385683_220000/LConn2
  220kV_Konin___Adamów_I_CN_171383831_220000_CN_216975352_220000/LConn3 -- T_171383831_220000;110000_Stacja_elektroenergetyczna_Adamów_220_110_kV/LConn3 -- 220kV_Adamów___Zgierz_CN_171383831_220000_CN_35366436_220000/LConn3 -- 220kV_Adamów___Zgierz_CN_171383831_220000_CN_101982559_220000/LConn3 -- 220kV_Adamów___Pabianice_CN_171383831_220000_CN_102165724_220000/LConn3 -- _CN_171383831_220000_CN_171385683_220000/LConn3 -- bus9/LConn1
  220kV_Konin___Adamów_I_CN_171383831_220000_CN_216975352_220000/RConn1 -- "T_216975352_220000;110000_Stacja_elektroenergetyczna_\"Konin\"_220_110_kV"/LConn1 -- 220kV_Konin___Sochaczew_CN_145037309_220000_CN_216975352_220000/LConn1 -- 220kV_Pątnów___Konin_I_CN_255284259_220000_CN_216975352_220000/LConn1 -- 220kV_Plewiska___Poznań_Południe_CN_131120723_220000_CN_216975352_220000/LConn1
  220kV_Konin___Adamów_I_CN_171383831_220000_CN_216975352_220000/RConn2 -- "T_216975352_220000;110000_Stacja_elektroenergetyczna_\"Konin\"_220_110_kV"/LConn2 -- 220kV_Konin___Sochaczew_CN_145037309_220000_CN_216975352_220000/LConn2 -- 220kV_Pątnów___Konin_I_CN_255284259_220000_CN_216975352_220000/LConn2 -- 220kV_Plewiska___Poznań_Południe_CN_131120723_220000_CN_216975352_220000/LConn2
  220kV_Konin___Adamów_I_CN_171383831_220000_CN_216975352_220000/RConn3 -- "T_216975352_220000;110000_Stacja_elektroenergetyczna_\"Konin\"_220_110_kV"/LConn3 -- 220kV_Konin___Sochaczew_CN_145037309_220000_CN_216975352_220000/LConn3 -- bus10/LConn1 -- 220kV_Pątnów___Konin_I_CN_255284259_220000_CN_216975352_220000/LConn3 -- 220kV_Plewiska___Poznań_Południe_CN_131120723_220000_CN_216975352_220000/LConn3
  220kV_Adamów___Zgierz_CN_171383831_220000_CN_35366436_220000/RConn1 -- "T_35366436_220000;110000_Stacja_elektroenergetyczna_\"Janów\"_220_110_kV"/LConn1 -- 220kV_Janów___Ołtarzew_CN_251239544_220000_CN_35366436_220000/LConn1 -- 220_kV_Pabianice___Janów_CN_35366436_220000_CN_102165724_220000/LConn1 -- 220kV_Rogowiec___Piotrków_CN_170316833_220000_CN_35366436_220000/LConn1
  220kV_Adamów___Zgierz_CN_171383831_220000_CN_35366436_220000/RConn2 -- "T_35366436_220000;110000_Stacja_elektroenergetyczna_\"Janów\"_220_110_kV"/LConn2 -- 220kV_Janów___Ołtarzew_CN_251239544_220000_CN_35366436_220000/LConn2 -- 220_kV_Pabianice___Janów_CN_35366436_220000_CN_102165724_220000/LConn2 -- 220kV_Rogowiec___Piotrków_CN_170316833_220000_CN_35366436_220000/LConn2
  220kV_Adamów___Zgierz_CN_171383831_220000_CN_35366436_220000/RConn3 -- "T_35366436_220000;110000_Stacja_elektroenergetyczna_\"Janów\"_220_110_kV"/LConn3 -- 220kV_Janów___Ołtarzew_CN_251239544_220000_CN_35366436_220000/LConn3 -- 220_kV_Pabianice___Janów_CN_35366436_220000_CN_102165724_220000/LConn3 -- bus11/LConn1 -- 220kV_Rogowiec___Piotrków_CN_170316833_220000_CN_35366436_220000/LConn3
  T_101982559_220000;110000_Stacja_elektroenergetyczna_„Zgierz”_220_110_kV/LConn1 -- 220kV_Adamów___Zgierz_CN_171383831_220000_CN_101982559_220000/RConn1
  T_101982559_220000;110000_Stacja_elektroenergetyczna_„Zgierz”_220_110_kV/LConn2 -- 220kV_Adamów___Zgierz_CN_171383831_220000_CN_101982559_220000/RConn2
  220kV_Adamów___Zgierz_CN_171383831_220000_CN_101982559_220000/RConn3 -- T_101982559_220000;110000_Stacja_elektroenergetyczna_„Zgierz”_220_110_kV/LConn3 -- bus12/LConn1
  220kV_Adamów___Pabianice_CN_171383831_220000_CN_102165724_220000/RConn1 -- "T_102165724_220000;110000_Stacja_elektroenergetyczna_\"Pabianice\"_220_110_kV"/LConn1 -- 220_kV_Pabianice___Janów_CN_35366436_220000_CN_102165724_220000/RConn1 -- 220kV_Rogowiec___Pabianice_CN_293484891_220000_CN_102165724_220000/LConn1
  220kV_Adamów___Pabianice_CN_171383831_220000_CN_102165724_220000/RConn2 -- "T_102165724_220000;110000_Stacja_elektroenergetyczna_\"Pabianice\"_220_110_kV"/LConn2 -- 220_kV_Pabianice___Janów_CN_35366436_220000_CN_102165724_220000/RConn2 -- 220kV_Rogowiec___Pabianice_CN_293484891_220000_CN_102165724_220000/LConn2
  220kV_Adamów___Pabianice_CN_171383831_220000_CN_102165724_220000/RConn3 -- "T_102165724_220000;110000_Stacja_elektroenergetyczna_\"Pabianice\"_220_110_kV"/LConn3 -- 220_kV_Pabianice___Janów_CN_35366436_220000_CN_102165724_220000/RConn3 -- bus13/LConn1 -- 220kV_Rogowiec___Pabianice_CN_293484891_220000_CN_102165724_220000/LConn3
  G_171385683_Elektrownia_Adamów/RConn1 -- _CN_171383831_220000_CN_171385683_220000/RConn1
  G_171385683_Elektrownia_Adamów/RConn2 -- _CN_171383831_220000_CN_171385683_220000/RConn2
  _CN_171383831_220000_CN_171385683_220000/RConn3 -- G_171385683_Elektrownia_Adamów/RConn3 -- bus14/LConn1
  220kV_Jasiniec___Gdańsk_I_CN_154838041_220000_CN_385098015_220000/LConn1 -- "T_154838041_400000;220000;110000_Stacja_elektroenergetyczna_\"Gdańsk_I\"_400_220_110_kV"/RConn1 -- 220kV_Gdańsk_I___Żydowo_CN_154838041_220000_CN_178838661_220000/LConn1 -- L_154838041/LConn1
  220kV_Jasiniec___Gdańsk_I_CN_154838041_220000_CN_385098015_220000/LConn2 -- "T_154838041_400000;220000;110000_Stacja_elektroenergetyczna_\"Gdańsk_I\"_400_220_110_kV"/RConn2 -- 220kV_Gdańsk_I___Żydowo_CN_154838041_220000_CN_178838661_220000/LConn2 -- L_154838041/LConn2
  220kV_Jasiniec___Gdańsk_I_CN_154838041_220000_CN_385098015_220000/LConn3 -- "T_154838041_400000;220000;110000_Stacja_elektroenergetyczna_\"Gdańsk_I\"_400_220_110_kV"/RConn3 -- 220kV_Gdańsk_I___Żydowo_CN_154838041_220000_CN_178838661_220000/LConn3 -- L_154838041/LConn3 -- bus15/LConn1
  220kV_Jasiniec___Gdańsk_I_CN_154838041_220000_CN_385098015_220000/RConn1 -- T_385098015__Stacja_elektroenergetyczna_400_110_kV_Pelplin/LConn1 -- 220kV_Jasiniec___Gdańsk_I_CN_385098015_220000_CN_46235456_220000/LConn1
  220kV_Jasiniec___Gdańsk_I_CN_154838041_220000_CN_385098015_220000/RConn2 -- T_385098015__Stacja_elektroenergetyczna_400_110_kV_Pelplin/LConn2 -- 220kV_Jasiniec___Gdańsk_I_CN_385098015_220000_CN_46235456_220000/LConn2
  220kV_Jasiniec___Gdańsk_I_CN_154838041_220000_CN_385098015_220000/RConn3 -- T_385098015__Stacja_elektroenergetyczna_400_110_kV_Pelplin/LConn3 -- 220kV_Jasiniec___Gdańsk_I_CN_385098015_220000_CN_46235456_220000/LConn3 -- bus16/LConn1
  220kV_Gdańsk_I___Żydowo_CN_154838041_220000_CN_178838661_220000/RConn1 -- "T_178838661_220000;110000_Stacja_elektroenergetyczna_\"Żydowo\"_220_110_kV"/LConn1 -- 220_kV_Dunowo___Żydowo_CN_178838661_220000_CN_175406958_220000/LConn1 -- 220kV_Piła_Krzewina___Żydowo_CN_178838661_220000_CN_238640596_220000/LConn1
  220kV_Gdańsk_I___Żydowo_CN_154838041_220000_CN_178838661_220000/RConn2 -- "T_178838661_220000;110000_Stacja_elektroenergetyczna_\"Żydowo\"_220_110_kV"/LConn2 -- 220_kV_Dunowo___Żydowo_CN_178838661_220000_CN_175406958_220000/LConn2 -- 220kV_Piła_Krzewina___Żydowo_CN_178838661_220000_CN_238640596_220000/LConn2
  220kV_Gdańsk_I___Żydowo_CN_154838041_220000_CN_178838661_220000/RConn3 -- "T_178838661_220000;110000_Stacja_elektroenergetyczna_\"Żydowo\"_220_110_kV"/LConn3 -- 220_kV_Dunowo___Żydowo_CN_178838661_220000_CN_175406958_220000/LConn3 -- 220kV_Piła_Krzewina___Żydowo_CN_178838661_220000_CN_238640596_220000/LConn3 -- bus17/LConn1
  220kV_Rogowiec___Piotrków_CN_170316833_220000_CN_293484891_220000/LConn1 -- T_170316833_220000;110000_Stacja_elektroenergetyczna_„Piotrków”_220_110_kV/LConn1 -- 220kV_Rogowiec___Piotrków_CN_170316833_220000_CN_35366436_220000/RConn1
  220kV_Rogowiec___Piotrków_CN_170316833_220000_CN_293484891_220000/LConn2 -- T_170316833_220000;110000_Stacja_elektroenergetyczna_„Piotrków”_220_110_kV/LConn2 -- 220kV_Rogowiec___Piotrków_CN_170316833_220000_CN_35366436_220000/RConn2
  220kV_Rogowiec___Piotrków_CN_170316833_220000_CN_293484891_220000/LConn3 -- T_170316833_220000;110000_Stacja_elektroenergetyczna_„Piotrków”_220_110_kV/LConn3 -- 220kV_Rogowiec___Piotrków_CN_170316833_220000_CN_35366436_220000/RConn3 -- bus18/LConn1
  220kV_Rogowiec___Piotrków_CN_170316833_220000_CN_293484891_220000/RConn1 -- "T_293484891_400000;220000_Stacja_elektroenergetyczna_\"Rogowiec\"_400_220_kV"/RConn1 -- 220kV_Rogowiec___Kopalnia_Bełchatów_[2__CN_155971668_220000_CN_293484891_220000/LConn1 -- 220kV_Rogowiec___Pabianice_CN_293484891_220000_CN_102165724_220000/RConn1 -- 220kV_Rogowiec___Joachimów_tor_2_CN_293484891_220000_CN_216060722_220000/LConn1 -- 220kV_Rogowiec___Joachimów_tor_2_CN_293484891_220000_CN_241842600_220000/LConn1 -- L_293484891/LConn1
  220kV_Rogowiec___Piotrków_CN_170316833_220000_CN_293484891_220000/RConn2 -- "T_293484891_400000;220000_Stacja_elektroenergetyczna_\"Rogowiec\"_400_220_kV"/RConn2 -- 220kV_Rogowiec___Kopalnia_Bełchatów_[2__CN_155971668_220000_CN_293484891_220000/LConn2 -- 220kV_Rogowiec___Pabianice_CN_293484891_220000_CN_102165724_220000/RConn2 -- 220kV_Rogowiec___Joachimów_tor_2_CN_293484891_220000_CN_216060722_220000/LConn2 -- 220kV_Rogowiec___Joachimów_tor_2_CN_293484891_220000_CN_241842600_220000/LConn2 -- L_293484891/LConn2
  220kV_Rogowiec___Piotrków_CN_170316833_220000_CN_293484891_220000/RConn3 -- "T_293484891_400000;220000_Stacja_elektroenergetyczna_\"Rogowiec\"_400_220_kV"/RConn3 -- 220kV_Rogowiec___Kopalnia_Bełchatów_[2__CN_155971668_220000_CN_293484891_220000/LConn3 -- 220kV_Rogowiec___Pabianice_CN_293484891_220000_CN_102165724_220000/RConn3 -- 220kV_Rogowiec___Joachimów_tor_2_CN_293484891_220000_CN_216060722_220000/LConn3 -- 220kV_Rogowiec___Joachimów_tor_2_CN_293484891_220000_CN_241842600_220000/LConn3 -- L_293484891/LConn3 -- bus19/LConn1
  220kV_Pątnów___Czerwonak_CN_255284259_220000_CN_180824706_220000/LConn1 -- "T_255284259_220000;110000_Stacja_elektroenergetyczna_\"Pątnów\"_220_110_kV"/LConn1 -- 220kV_Pątnów___Konin_I_CN_255284259_220000_CN_216975352_220000/RConn1 -- 220kV_Pątnów___Podolszyce_CN_255284259_220000_CN_29115701_220000/LConn1 -- 220kV_Pątnów___Podolszyce_CN_255284259_220000_CN_171992870_220000/LConn1 -- 220kV_Pątnów___Włocławek_Azoty_CN_255284259_220000_CN_72879943_220000/LConn1 -- 220kV_Pątnów___Bydgoszcz_Jasiniec_tor_I_CN_255284259_220000_CN_46235456_220000/LConn1
  220kV_Pątnów___Czerwonak_CN_255284259_220000_CN_180824706_220000/LConn2 -- "T_255284259_220000;110000_Stacja_elektroenergetyczna_\"Pątnów\"_220_110_kV"/LConn2 -- 220kV_Pątnów___Konin_I_CN_255284259_220000_CN_216975352_220000/RConn2 -- 220kV_Pątnów___Podolszyce_CN_255284259_220000_CN_29115701_220000/LConn2 -- 220kV_Pątnów___Podolszyce_CN_255284259_220000_CN_171992870_220000/LConn2 -- 220kV_Pątnów___Włocławek_Azoty_CN_255284259_220000_CN_72879943_220000/LConn2 -- 220kV_Pątnów___Bydgoszcz_Jasiniec_tor_I_CN_255284259_220000_CN_46235456_220000/LConn2
  220kV_Pątnów___Czerwonak_CN_255284259_220000_CN_180824706_220000/LConn3 -- "T_255284259_220000;110000_Stacja_elektroenergetyczna_\"Pątnów\"_220_110_kV"/LConn3 -- 220kV_Pątnów___Konin_I_CN_255284259_220000_CN_216975352_220000/RConn3 -- 220kV_Pątnów___Podolszyce_CN_255284259_220000_CN_29115701_220000/LConn3 -- 220kV_Pątnów___Podolszyce_CN_255284259_220000_CN_171992870_220000/LConn3 -- 220kV_Pątnów___Włocławek_Azoty_CN_255284259_220000_CN_72879943_220000/LConn3 -- 220kV_Pątnów___Bydgoszcz_Jasiniec_tor_I_CN_255284259_220000_CN_46235456_220000/LConn3 -- bus20/LConn1
  220kV_Pątnów___Czerwonak_CN_255284259_220000_CN_180824706_220000/RConn1 -- "T_180824706_220000;110000_Stacja_elektroenergetyczna_\"Czerwonak\"_220_110_kV"/LConn1 -- 220kV_Plewiska___Czerwonak_CN_180824706_220000_CN_32036484_220000/LConn1
  220kV_Pątnów___Czerwonak_CN_255284259_220000_CN_180824706_220000/RConn2 -- "T_180824706_220000;110000_Stacja_elektroenergetyczna_\"Czerwonak\"_220_110_kV"/LConn2 -- 220kV_Plewiska___Czerwonak_CN_180824706_220000_CN_32036484_220000/LConn2
  220kV_Pątnów___Czerwonak_CN_255284259_220000_CN_180824706_220000/RConn3 -- "T_180824706_220000;110000_Stacja_elektroenergetyczna_\"Czerwonak\"_220_110_kV"/LConn3 -- 220kV_Plewiska___Czerwonak_CN_180824706_220000_CN_32036484_220000/LConn3 -- bus21/LConn1
  220kV_Pątnów___Podolszyce_CN_255284259_220000_CN_29115701_220000/RConn1 -- "T_29115701_220000;110000_Stacja_elektroenergetyczna_\"Mory\"_220_110kV"/LConn1 -- 220_kV_Mory___Miłosna_CN_29115701_220000_CN_99593626_220000/LConn1 -- 220kV_Mory___Piaseczno_CN_29115701_220000_CN_29098336_220000/LConn1 -- 220kV_Mory___Piaseczno_CN_29115701_220000_CN_173582810_220000/LConn1 -- 220kV_Ołtarzew___Mory_CN_251239544_220000_CN_29115701_220000/LConn1 -- 220kV_Mory___Towarowa_CN_89434732_220000_CN_29115701_220000/LConn1
  220kV_Pątnów___Podolszyce_CN_255284259_220000_CN_29115701_220000/RConn2 -- "T_29115701_220000;110000_Stacja_elektroenergetyczna_\"Mory\"_220_110kV"/LConn2 -- 220_kV_Mory___Miłosna_CN_29115701_220000_CN_99593626_220000/LConn2 -- 220kV_Mory___Piaseczno_CN_29115701_220000_CN_29098336_220000/LConn2 -- 220kV_Mory___Piaseczno_CN_29115701_220000_CN_173582810_220000/LConn2 -- 220kV_Ołtarzew___Mory_CN_251239544_220000_CN_29115701_220000/LConn2 -- 220kV_Mory___Towarowa_CN_89434732_220000_CN_29115701_220000/LConn2
  220kV_Pątnów___Podolszyce_CN_255284259_220000_CN_29115701_220000/RConn3 -- "T_29115701_220000;110000_Stacja_elektroenergetyczna_\"Mory\"_220_110kV"/LConn3 -- 220_kV_Mory___Miłosna_CN_29115701_220000_CN_99593626_220000/LConn3 -- 220kV_Mory___Piaseczno_CN_29115701_220000_CN_29098336_220000/LConn3 -- 220kV_Mory___Piaseczno_CN_29115701_220000_CN_173582810_220000/LConn3 -- bus22/LConn1 -- 220kV_Ołtarzew___Mory_CN_251239544_220000_CN_29115701_220000/LConn3 -- 220kV_Mory___Towarowa_CN_89434732_220000_CN_29115701_220000/LConn3
  "T_171992870_220000;110000_Stacja_elektroenergetyczna_\"Podolszyce\"_220_110kV"/LConn1 -- 220kV_Pątnów___Podolszyce_CN_255284259_220000_CN_171992870_220000/RConn1
  "T_171992870_220000;110000_Stacja_elektroenergetyczna_\"Podolszyce\"_220_110kV"/LConn2 -- 220kV_Pątnów___Podolszyce_CN_255284259_220000_CN_171992870_220000/RConn2
  220kV_Pątnów___Podolszyce_CN_255284259_220000_CN_171992870_220000/RConn3 -- "T_171992870_220000;110000_Stacja_elektroenergetyczna_\"Podolszyce\"_220_110kV"/LConn3 -- bus23/LConn1
  220kV_Pątnów___Włocławek_Azoty_CN_255284259_220000_CN_72879943_220000/RConn1 -- "T_72879943_220000;110000_Stacja_elektroenergetyczna_\"Włocławek_Azoty\"_220_110_kV"/LConn1 -- 220kV_Włocławek___Olsztyn_CN_101915790_220000_CN_72879943_220000/LConn1 -- 220kV_Toruń_Elana___Włocławek_Azoty_CN_72879943_220000_CN_143484238_220000/LConn1
  220kV_Pątnów___Włocławek_Azoty_CN_255284259_220000_CN_72879943_220000/RConn2 -- "T_72879943_220000;110000_Stacja_elektroenergetyczna_\"Włocławek_Azoty\"_220_110_kV"/LConn2 -- 220kV_Włocławek___Olsztyn_CN_101915790_220000_CN_72879943_220000/LConn2 -- 220kV_Toruń_Elana___Włocławek_Azoty_CN_72879943_220000_CN_143484238_220000/LConn2
  220kV_Pątnów___Włocławek_Azoty_CN_255284259_220000_CN_72879943_220000/RConn3 -- "T_72879943_220000;110000_Stacja_elektroenergetyczna_\"Włocławek_Azoty\"_220_110_kV"/LConn3 -- 220kV_Włocławek___Olsztyn_CN_101915790_220000_CN_72879943_220000/LConn3 -- 220kV_Toruń_Elana___Włocławek_Azoty_CN_72879943_220000_CN_143484238_220000/LConn3 -- bus24/LConn1
  220kV_Pątnów___Bydgoszcz_Jasiniec_tor_I_CN_255284259_220000_CN_46235456_220000/RConn1 -- "T_46235456_220000;110000_Stacja_elektroenergetyczna_\"Jasiniec\"_220_110_kV"/LConn1 -- 220_kV_Bydgoszcz_Jasiniec___Grudziądz_Węgrowo_CN_46092396_220000_CN_46235456_220000/LConn1 -- 220kV_Jasiniec___Gdańsk_I_CN_385098015_220000_CN_46235456_220000/RConn1 -- 220kV_Jasiniec___Bydgoszcz_Zachód_CN_46235456_220000_CN_255293400_220000/LConn1
  220kV_Pątnów___Bydgoszcz_Jasiniec_tor_I_CN_255284259_220000_CN_46235456_220000/RConn2 -- "T_46235456_220000;110000_Stacja_elektroenergetyczna_\"Jasiniec\"_220_110_kV"/LConn2 -- 220_kV_Bydgoszcz_Jasiniec___Grudziądz_Węgrowo_CN_46092396_220000_CN_46235456_220000/LConn2 -- 220kV_Jasiniec___Gdańsk_I_CN_385098015_220000_CN_46235456_220000/RConn2 -- 220kV_Jasiniec___Bydgoszcz_Zachód_CN_46235456_220000_CN_255293400_220000/LConn2
  220kV_Pątnów___Bydgoszcz_Jasiniec_tor_I_CN_255284259_220000_CN_46235456_220000/RConn3 -- "T_46235456_220000;110000_Stacja_elektroenergetyczna_\"Jasiniec\"_220_110_kV"/LConn3 -- 220_kV_Bydgoszcz_Jasiniec___Grudziądz_Węgrowo_CN_46092396_220000_CN_46235456_220000/LConn3 -- 220kV_Jasiniec___Gdańsk_I_CN_385098015_220000_CN_46235456_220000/RConn3 -- 220kV_Jasiniec___Bydgoszcz_Zachód_CN_46235456_220000_CN_255293400_220000/LConn3 -- bus25/LConn1
  220kV_Żar___Bujaków_CN_44389929_220000_CN_98611253_220000/LConn1 -- "T_44389929_220000_Stacja_elektroenergetyczna_\"Bujaków\"_220kV"/LConn1 -- 220kV_Bujaków___Komorowice_CN_44389929_220000_CN_98634956_220000/LConn1 -- 220kV_Bujaków___Komorowice_CN_44389929_220000_CN_291375946_220000/LConn1 -- 220kV_Bujaków___Komorowice_CN_44389929_220000_CN_135598292_220000/LConn1 -- 220kV_Bujaków___Komorowice_CN_44389929_220000_CN_255232597_220000/LConn1 -- 220kV_Bujaków___Komorowice_CN_44389929_220000_CN_133537926_220000/LConn1 -- 220kV_Bujaków___Komorowice_CN_44389929_220000_CN_184899160_220000/LConn1 -- 220kV_Bujaków___Komorowice_CN_44389929_220000_CN_139452056_220000/LConn1 -- 220kV_Bujaków___Komorowice_CN_44389929_220000_CN_183945016_220000/LConn1
  220kV_Żar___Bujaków_CN_44389929_220000_CN_98611253_220000/LConn2 -- "T_44389929_220000_Stacja_elektroenergetyczna_\"Bujaków\"_220kV"/LConn2 -- 220kV_Bujaków___Komorowice_CN_44389929_220000_CN_98634956_220000/LConn2 -- 220kV_Bujaków___Komorowice_CN_44389929_220000_CN_291375946_220000/LConn2 -- 220kV_Bujaków___Komorowice_CN_44389929_220000_CN_135598292_220000/LConn2 -- 220kV_Bujaków___Komorowice_CN_44389929_220000_CN_255232597_220000/LConn2 -- 220kV_Bujaków___Komorowice_CN_44389929_220000_CN_133537926_220000/LConn2 -- 220kV_Bujaków___Komorowice_CN_44389929_220000_CN_184899160_220000/LConn2 -- 220kV_Bujaków___Komorowice_CN_44389929_220000_CN_139452056_220000/LConn2 -- 220kV_Bujaków___Komorowice_CN_44389929_220000_CN_183945016_220000/LConn2
  220kV_Żar___Bujaków_CN_44389929_220000_CN_98611253_220000/LConn3 -- "T_44389929_220000_Stacja_elektroenergetyczna_\"Bujaków\"_220kV"/LConn3 -- 220kV_Bujaków___Komorowice_CN_44389929_220000_CN_98634956_220000/LConn3 -- 220kV_Bujaków___Komorowice_CN_44389929_220000_CN_291375946_220000/LConn3 -- 220kV_Bujaków___Komorowice_CN_44389929_220000_CN_135598292_220000/LConn3 -- 220kV_Bujaków___Komorowice_CN_44389929_220000_CN_255232597_220000/LConn3 -- 220kV_Bujaków___Komorowice_CN_44389929_220000_CN_133537926_220000/LConn3 -- 220kV_Bujaków___Komorowice_CN_44389929_220000_CN_184899160_220000/LConn3 -- 220kV_Bujaków___Komorowice_CN_44389929_220000_CN_139452056_220000/LConn3 -- 220kV_Bujaków___Komorowice_CN_44389929_220000_CN_183945016_220000/LConn3 -- bus26/LConn1
  G_98611253_Elektrownia_szczytowo_pompowa_Porąbka_Żar/RConn1 -- 220kV_Żar___Bujaków_CN_44389929_220000_CN_98611253_220000/RConn1
  G_98611253_Elektrownia_szczytowo_pompowa_Porąbka_Żar/RConn2 -- 220kV_Żar___Bujaków_CN_44389929_220000_CN_98611253_220000/RConn2
  220kV_Żar___Bujaków_CN_44389929_220000_CN_98611253_220000/RConn3 -- G_98611253_Elektrownia_szczytowo_pompowa_Porąbka_Żar/RConn3 -- bus27/LConn1
  "T_98634956_220000;110000_Stacja_elektroenergetyczna_\"Komorowice\"_220_110_kV"/LConn1 -- 220kV_Bujaków___Komorowice_CN_44389929_220000_CN_98634956_220000/RConn1
  "T_98634956_220000;110000_Stacja_elektroenergetyczna_\"Komorowice\"_220_110_kV"/LConn2 -- 220kV_Bujaków___Komorowice_CN_44389929_220000_CN_98634956_220000/RConn2
  220kV_Bujaków___Komorowice_CN_44389929_220000_CN_98634956_220000/RConn3 -- "T_98634956_220000;110000_Stacja_elektroenergetyczna_\"Komorowice\"_220_110_kV"/LConn3 -- bus28/LConn1
  T_291375946__Stacja_elektroenergetyczna_„Czeczot”_220_110_kV/LConn1 -- 220kV_Bujaków___Komorowice_CN_44389929_220000_CN_291375946_220000/RConn1
  T_291375946__Stacja_elektroenergetyczna_„Czeczot”_220_110_kV/LConn2 -- 220kV_Bujaków___Komorowice_CN_44389929_220000_CN_291375946_220000/RConn2
  220kV_Bujaków___Komorowice_CN_44389929_220000_CN_291375946_220000/RConn3 -- T_291375946__Stacja_elektroenergetyczna_„Czeczot”_220_110_kV/LConn3 -- bus29/LConn1
  T_135598292_220000;110000_Stacja_elektroenergetyczna_„Poręba”_220_110_kV/LConn1 -- 220kV_Bujaków___Komorowice_CN_44389929_220000_CN_135598292_220000/RConn1
  T_135598292_220000;110000_Stacja_elektroenergetyczna_„Poręba”_220_110_kV/LConn2 -- 220kV_Bujaków___Komorowice_CN_44389929_220000_CN_135598292_220000/RConn2
  220kV_Bujaków___Komorowice_CN_44389929_220000_CN_135598292_220000/RConn3 -- T_135598292_220000;110000_Stacja_elektroenergetyczna_„Poręba”_220_110_kV/LConn3 -- bus30/LConn1
  "T_255232597_220000;110000_Stacja_elektroenergetyczna_\"Bieruń\"_220_110_kV"/LConn1 -- 220kV_Bujaków___Komorowice_CN_44389929_220000_CN_255232597_220000/RConn1
  "T_255232597_220000;110000_Stacja_elektroenergetyczna_\"Bieruń\"_220_110_kV"/LConn2 -- 220kV_Bujaków___Komorowice_CN_44389929_220000_CN_255232597_220000/RConn2
  220kV_Bujaków___Komorowice_CN_44389929_220000_CN_255232597_220000/RConn3 -- "T_255232597_220000;110000_Stacja_elektroenergetyczna_\"Bieruń\"_220_110_kV"/LConn3 -- bus31/LConn1
  220kV_Bujaków___Komorowice_CN_44389929_220000_CN_133537926_220000/RConn1 -- T_133537926_220000_Stacja_elektroenergetyczna_„Byczyna”_220_kV/LConn1 -- 220kV_BLOK_1___Byczyna_CN_133537926_220000_CN_105864304_220000/LConn1 -- 220kV_Łagisza___Byczyna___Halemba_CN_133537926_220000_CN_183259405_220000/LConn1 -- 220kV_Łagisza___Byczyna___Halemba_CN_133537926_220000_CN_183945016_220000/LConn1 -- 220kV_Łagisza___Byczyna___Halemba_CN_133537926_220000_CN_66161634_220000/LConn1 -- 220kV_Łagisza___Byczyna___Halemba_CN_133537926_220000_CN_29139402_220000/LConn1 -- 220kV_Byczyna___Skawina_CN_133537926_220000_CN_187420591_220000/RConn1 -- 220kV_Byczyna___Skawina_CN_133537926_220000_CN_179864449_220000/RConn1 -- 220kV_Byczyna___Jamki_CN_40946790_220000_CN_133537926_220000/LConn1
  220kV_Bujaków___Komorowice_CN_44389929_220000_CN_133537926_220000/RConn2 -- T_133537926_220000_Stacja_elektroenergetyczna_„Byczyna”_220_kV/LConn2 -- 220kV_BLOK_1___Byczyna_CN_133537926_220000_CN_105864304_220000/LConn2 -- 220kV_Łagisza___Byczyna___Halemba_CN_133537926_220000_CN_183259405_220000/LConn2 -- 220kV_Łagisza___Byczyna___Halemba_CN_133537926_220000_CN_183945016_220000/LConn2 -- 220kV_Łagisza___Byczyna___Halemba_CN_133537926_220000_CN_66161634_220000/LConn2 -- 220kV_Łagisza___Byczyna___Halemba_CN_133537926_220000_CN_29139402_220000/LConn2 -- 220kV_Byczyna___Skawina_CN_133537926_220000_CN_187420591_220000/RConn2 -- 220kV_Byczyna___Skawina_CN_133537926_220000_CN_179864449_220000/RConn2 -- 220kV_Byczyna___Jamki_CN_40946790_220000_CN_133537926_220000/LConn2
  220kV_Bujaków___Komorowice_CN_44389929_220000_CN_133537926_220000/RConn3 -- T_133537926_220000_Stacja_elektroenergetyczna_„Byczyna”_220_kV/LConn3 -- 220kV_BLOK_1___Byczyna_CN_133537926_220000_CN_105864304_220000/LConn3 -- 220kV_Łagisza___Byczyna___Halemba_CN_133537926_220000_CN_183259405_220000/LConn3 -- 220kV_Łagisza___Byczyna___Halemba_CN_133537926_220000_CN_183945016_220000/LConn3 -- 220kV_Łagisza___Byczyna___Halemba_CN_133537926_220000_CN_66161634_220000/LConn3 -- 220kV_Łagisza___Byczyna___Halemba_CN_133537926_220000_CN_29139402_220000/LConn3 -- bus32/LConn1 -- 220kV_Byczyna___Skawina_CN_133537926_220000_CN_187420591_220000/RConn3 -- 220kV_Byczyna___Skawina_CN_133537926_220000_CN_179864449_220000/RConn3 -- 220kV_Byczyna___Jamki_CN_40946790_220000_CN_133537926_220000/LConn3
  T_184899160_220000;110000_Stacja_elektroenergetyczna_„Moszczenica”_220_110_kV/LConn1 -- 220kV_Bujaków___Komorowice_CN_44389929_220000_CN_184899160_220000/RConn1
  T_184899160_220000;110000_Stacja_elektroenergetyczna_„Moszczenica”_220_110_kV/LConn2 -- 220kV_Bujaków___Komorowice_CN_44389929_220000_CN_184899160_220000/RConn2
  220kV_Bujaków___Komorowice_CN_44389929_220000_CN_184899160_220000/RConn3 -- T_184899160_220000;110000_Stacja_elektroenergetyczna_„Moszczenica”_220_110_kV/LConn3 -- bus33/LConn1
  220kV_Bujaków___Komorowice_CN_44389929_220000_CN_139452056_220000/RConn1 -- T_139452056_400000;220000;110000_Stacja_elektroenergetyczna_„Wielopole”_400_220_110_kV/RConn1 -- 220kV_Wielopole___Blachownia_CN_185454704_220000_CN_139452056_220000/LConn1 -- L_139452056/LConn1
  220kV_Bujaków___Komorowice_CN_44389929_220000_CN_139452056_220000/RConn2 -- T_139452056_400000;220000;110000_Stacja_elektroenergetyczna_„Wielopole”_400_220_110_kV/RConn2 -- 220kV_Wielopole___Blachownia_CN_185454704_220000_CN_139452056_220000/LConn2 -- L_139452056/LConn2
  220kV_Bujaków___Komorowice_CN_44389929_220000_CN_139452056_220000/RConn3 -- T_139452056_400000;220000;110000_Stacja_elektroenergetyczna_„Wielopole”_400_220_110_kV/RConn3 -- 220kV_Wielopole___Blachownia_CN_185454704_220000_CN_139452056_220000/LConn3 -- L_139452056/LConn3 -- bus34/LConn1
  220kV_Bujaków___Komorowice_CN_44389929_220000_CN_183945016_220000/RConn1 -- "T_183945016_220000;110000_Stacja_elektroenergetyczna_\"Kopanina\"_220_110_kV"/LConn1 -- 220kV_Łagisza___Byczyna___Halemba_CN_133537926_220000_CN_183945016_220000/RConn1
  220kV_Bujaków___Komorowice_CN_44389929_220000_CN_183945016_220000/RConn2 -- "T_183945016_220000;110000_Stacja_elektroenergetyczna_\"Kopanina\"_220_110_kV"/LConn2 -- 220kV_Łagisza___Byczyna___Halemba_CN_133537926_220000_CN_183945016_220000/RConn2
  220kV_Bujaków___Komorowice_CN_44389929_220000_CN_183945016_220000/RConn3 -- "T_183945016_220000;110000_Stacja_elektroenergetyczna_\"Kopanina\"_220_110_kV"/LConn3 -- 220kV_Łagisza___Byczyna___Halemba_CN_133537926_220000_CN_183945016_220000/RConn3 -- bus35/LConn1
  "T_135175732__Stacja_elektroenergetyczna_\"Biskupice\"_220_110kV"/LConn1 -- 220kV_Świebodzice___Klecina_odg_Biskupice_CN_135175732_220000_CN_179138441_220000/LConn1
  "T_135175732__Stacja_elektroenergetyczna_\"Biskupice\"_220_110kV"/LConn2 -- 220kV_Świebodzice___Klecina_odg_Biskupice_CN_135175732_220000_CN_179138441_220000/LConn2
  220kV_Świebodzice___Klecina_odg_Biskupice_CN_135175732_220000_CN_179138441_220000/LConn3 -- "T_135175732__Stacja_elektroenergetyczna_\"Biskupice\"_220_110kV"/LConn3 -- bus36/LConn1
  220kV_Świebodzice___Klecina_odg_Biskupice_CN_135175732_220000_CN_179138441_220000/RConn1 -- T_179138441_220000;110000_Stacja_elektroenergetyczna_„Świebodzice”_220_110_kV/LConn1 -- _CN_179138441_220000_CN_276291999_220000/LConn1 -- 220kV_Mikułowa___Swiebodzice_CN_111615226_220000_CN_179138441_220000/LConn1 -- 220kV_Boguszów___Świebodzice_CN_177749653_220000_CN_179138441_220000/LConn1
  220kV_Świebodzice___Klecina_odg_Biskupice_CN_135175732_220000_CN_179138441_220000/RConn2 -- T_179138441_220000;110000_Stacja_elektroenergetyczna_„Świebodzice”_220_110_kV/LConn2 -- _CN_179138441_220000_CN_276291999_220000/LConn2 -- 220kV_Mikułowa___Swiebodzice_CN_111615226_220000_CN_179138441_220000/LConn2 -- 220kV_Boguszów___Świebodzice_CN_177749653_220000_CN_179138441_220000/LConn2
  220kV_Świebodzice___Klecina_odg_Biskupice_CN_135175732_220000_CN_179138441_220000/RConn3 -- T_179138441_220000;110000_Stacja_elektroenergetyczna_„Świebodzice”_220_110_kV/LConn3 -- _CN_179138441_220000_CN_276291999_220000/LConn3 -- bus37/LConn1 -- 220kV_Mikułowa___Swiebodzice_CN_111615226_220000_CN_179138441_220000/LConn3 -- 220kV_Boguszów___Świebodzice_CN_177749653_220000_CN_179138441_220000/LConn3
  220kV_Leśniów___Żukowice_CN_180535363_220000_CN_158232924_220000/RConn1 -- "T_180535363_220000;110000_Stacja_elektroenergetyczna_\"Żukowice\"_220_110_kV"/LConn1 -- 220kV_Żukowice___Polkowice_CN_180535363_220000_CN_180542657_220000/LConn1
  220kV_Leśniów___Żukowice_CN_180535363_220000_CN_158232924_220000/RConn2 -- "T_180535363_220000;110000_Stacja_elektroenergetyczna_\"Żukowice\"_220_110_kV"/LConn2 -- 220kV_Żukowice___Polkowice_CN_180535363_220000_CN_180542657_220000/LConn2
  220kV_Leśniów___Żukowice_CN_180535363_220000_CN_158232924_220000/RConn3 -- "T_180535363_220000;110000_Stacja_elektroenergetyczna_\"Żukowice\"_220_110_kV"/LConn3 -- 220kV_Żukowice___Polkowice_CN_180535363_220000_CN_180542657_220000/LConn3 -- bus38/LConn1
  220kV_Żukowice___Polkowice_CN_180535363_220000_CN_180542657_220000/RConn1 -- "T_180542657_220000;110000_Stacja_elektroenergetyczna_\"Polkowice\"_220_110_kV"/LConn1 -- 220kV_Plewiska___Leszno_CN_32036484_220000_CN_180542657_220000/LConn1 -- 220kV_Mikułowa___Polkowice_CN_180542657_220000_CN_111615226_220000/LConn1
  220kV_Żukowice___Polkowice_CN_180535363_220000_CN_180542657_220000/RConn2 -- "T_180542657_220000;110000_Stacja_elektroenergetyczna_\"Polkowice\"_220_110_kV"/LConn2 -- 220kV_Plewiska___Leszno_CN_32036484_220000_CN_180542657_220000/LConn2 -- 220kV_Mikułowa___Polkowice_CN_180542657_220000_CN_111615226_220000/LConn2
  220kV_Żukowice___Polkowice_CN_180535363_220000_CN_180542657_220000/RConn3 -- "T_180542657_220000;110000_Stacja_elektroenergetyczna_\"Polkowice\"_220_110_kV"/LConn3 -- 220kV_Plewiska___Leszno_CN_32036484_220000_CN_180542657_220000/LConn3 -- 220kV_Mikułowa___Polkowice_CN_180542657_220000_CN_111615226_220000/LConn3 -- bus39/LConn1
  220kV_Krajnik___Morzyczyn_CN_32943179_220000_CN_39428977_220000/RConn1 -- "T_32943179_400000;220000;110000_Stacja_elektroenergetyczna_\"Morzyczyn\"_400_220_110_kV"/RConn1 -- 220kV_Morzyczyn___Police_CN_32943179_220000_CN_165763717_220000/LConn1 -- L_32943179/LConn1
  220kV_Krajnik___Morzyczyn_CN_32943179_220000_CN_39428977_220000/RConn2 -- "T_32943179_400000;220000;110000_Stacja_elektroenergetyczna_\"Morzyczyn\"_400_220_110_kV"/RConn2 -- 220kV_Morzyczyn___Police_CN_32943179_220000_CN_165763717_220000/LConn2 -- L_32943179/LConn2
  220kV_Krajnik___Morzyczyn_CN_32943179_220000_CN_39428977_220000/RConn3 -- "T_32943179_400000;220000;110000_Stacja_elektroenergetyczna_\"Morzyczyn\"_400_220_110_kV"/RConn3 -- 220kV_Morzyczyn___Police_CN_32943179_220000_CN_165763717_220000/LConn3 -- L_32943179/LConn3 -- bus40/LConn1
  220kV_Morzyczyn___Police_CN_32943179_220000_CN_165763717_220000/RConn1 -- "T_165763717__Stacja_elektroenergetyczna_\"Police\"_220_110kV"/LConn1 -- 220kV_Glinki___Police_CN_165763717_220000_CN_40062974_220000/LConn1
  220kV_Morzyczyn___Police_CN_32943179_220000_CN_165763717_220000/RConn2 -- "T_165763717__Stacja_elektroenergetyczna_\"Police\"_220_110kV"/LConn2 -- 220kV_Glinki___Police_CN_165763717_220000_CN_40062974_220000/LConn2
  220kV_Morzyczyn___Police_CN_32943179_220000_CN_165763717_220000/RConn3 -- "T_165763717__Stacja_elektroenergetyczna_\"Police\"_220_110kV"/LConn3 -- 220kV_Glinki___Police_CN_165763717_220000_CN_40062974_220000/LConn3 -- bus41/LConn1
  220kV_Plewiska___Poznań_Południe_CN_131120723_220000_CN_32036484_220000/LConn1 -- T_131120723_220000;110000_Stacja_elektroenergetyczna_220_110_kV_Poznań_Południe/LConn1 -- 220kV_Plewiska___Poznań_Południe_CN_131120723_220000_CN_216975352_220000/RConn1
  220kV_Plewiska___Poznań_Południe_CN_131120723_220000_CN_32036484_220000/LConn2 -- T_131120723_220000;110000_Stacja_elektroenergetyczna_220_110_kV_Poznań_Południe/LConn2 -- 220kV_Plewiska___Poznań_Południe_CN_131120723_220000_CN_216975352_220000/RConn2
  220kV_Plewiska___Poznań_Południe_CN_131120723_220000_CN_32036484_220000/LConn3 -- T_131120723_220000;110000_Stacja_elektroenergetyczna_220_110_kV_Poznań_Południe/LConn3 -- 220kV_Plewiska___Poznań_Południe_CN_131120723_220000_CN_216975352_220000/RConn3 -- bus42/LConn1
  220kV_Plewiska___Poznań_Południe_CN_131120723_220000_CN_32036484_220000/RConn1 -- "T_32036484_400000;220000;110000_Stacja_elektroenergetyczna_\"Plewiska\"_400_220_110_kV"/RConn1 -- 220kV_Plewiska___Czerwonak_CN_180824706_220000_CN_32036484_220000/RConn1 -- 220kV_Plewiska___Leszno_CN_32036484_220000_CN_180542657_220000/RConn1 -- 220kV_Plewiska___Leszno_CN_32036484_220000_CN_148197330_220000/LConn1 -- 220kV_Plewiska___Piła_Krzewina_CN_32036484_220000_CN_238640596_220000/LConn1 -- L_32036484/LConn1
  220kV_Plewiska___Poznań_Południe_CN_131120723_220000_CN_32036484_220000/RConn2 -- "T_32036484_400000;220000;110000_Stacja_elektroenergetyczna_\"Plewiska\"_400_220_110_kV"/RConn2 -- 220kV_Plewiska___Czerwonak_CN_180824706_220000_CN_32036484_220000/RConn2 -- 220kV_Plewiska___Leszno_CN_32036484_220000_CN_180542657_220000/RConn2 -- 220kV_Plewiska___Leszno_CN_32036484_220000_CN_148197330_220000/LConn2 -- 220kV_Plewiska___Piła_Krzewina_CN_32036484_220000_CN_238640596_220000/LConn2 -- L_32036484/LConn2
  220kV_Plewiska___Poznań_Południe_CN_131120723_220000_CN_32036484_220000/RConn3 -- "T_32036484_400000;220000;110000_Stacja_elektroenergetyczna_\"Plewiska\"_400_220_110_kV"/RConn3 -- 220kV_Plewiska___Czerwonak_CN_180824706_220000_CN_32036484_220000/RConn3 -- 220kV_Plewiska___Leszno_CN_32036484_220000_CN_180542657_220000/RConn3 -- 220kV_Plewiska___Leszno_CN_32036484_220000_CN_148197330_220000/LConn3 -- 220kV_Plewiska___Piła_Krzewina_CN_32036484_220000_CN_238640596_220000/LConn3 -- L_32036484/LConn3 -- bus43/LConn1
  "T_155971668_220000;110000_Stacja_elektroenergetyczna_\"Kopalnia_Bełchatów\"_220_110kV"/LConn1 -- 220kV_Rogowiec___Kopalnia_Bełchatów_[2__CN_155971668_220000_CN_293484891_220000/RConn1
  "T_155971668_220000;110000_Stacja_elektroenergetyczna_\"Kopalnia_Bełchatów\"_220_110kV"/LConn2 -- 220kV_Rogowiec___Kopalnia_Bełchatów_[2__CN_155971668_220000_CN_293484891_220000/RConn2
  220kV_Rogowiec___Kopalnia_Bełchatów_[2__CN_155971668_220000_CN_293484891_220000/RConn3 -- "T_155971668_220000;110000_Stacja_elektroenergetyczna_\"Kopalnia_Bełchatów\"_220_110kV"/LConn3 -- bus44/LConn1
  T_173613665_220000;110000_Stacja_elektroenergetyczna_„Zamość”_220_110_kV/LConn1 -- 220kV_Mokre___Zamość_CN_173613665_220000_CN_170368942_220000/LConn1
  T_173613665_220000;110000_Stacja_elektroenergetyczna_„Zamość”_220_110_kV/LConn2 -- 220kV_Mokre___Zamość_CN_173613665_220000_CN_170368942_220000/LConn2
  220kV_Mokre___Zamość_CN_173613665_220000_CN_170368942_220000/LConn3 -- T_173613665_220000;110000_Stacja_elektroenergetyczna_„Zamość”_220_110_kV/LConn3 -- bus45/LConn1
  220kV_Mokre___Zamość_CN_173613665_220000_CN_170368942_220000/RConn1 -- T_170368942_220000;110000_Stacja_elektroenergetyczna_„Mokre”_220_110_kV/LConn1 -- 220kV_Mokre___Chełm_CN_194903381_220000_CN_170368942_220000/LConn1
  220kV_Mokre___Zamość_CN_173613665_220000_CN_170368942_220000/RConn2 -- T_170368942_220000;110000_Stacja_elektroenergetyczna_„Mokre”_220_110_kV/LConn2 -- 220kV_Mokre___Chełm_CN_194903381_220000_CN_170368942_220000/LConn2
  220kV_Mokre___Zamość_CN_173613665_220000_CN_170368942_220000/RConn3 -- T_170368942_220000;110000_Stacja_elektroenergetyczna_„Mokre”_220_110_kV/LConn3 -- 220kV_Mokre___Chełm_CN_194903381_220000_CN_170368942_220000/LConn3 -- bus46/LConn1
  220kV_Byczyna___Jamki_CN_40946790_220000_CN_66051759_220000/LConn1 -- "T_40946790_220000;110000_Stacja_elektroenergetyczna_\"Jamki\"_220_110kV"/LConn1 -- 220kV_Byczyna___Jamki_CN_40946790_220000_CN_133537926_220000/RConn1 -- 220kV_Łagisza___Jamki_CN_40946790_220000_CN_66161634_220000/LConn1
  220kV_Byczyna___Jamki_CN_40946790_220000_CN_66051759_220000/LConn2 -- "T_40946790_220000;110000_Stacja_elektroenergetyczna_\"Jamki\"_220_110kV"/LConn2 -- 220kV_Byczyna___Jamki_CN_40946790_220000_CN_133537926_220000/RConn2 -- 220kV_Łagisza___Jamki_CN_40946790_220000_CN_66161634_220000/LConn2
  220kV_Byczyna___Jamki_CN_40946790_220000_CN_66051759_220000/LConn3 -- "T_40946790_220000;110000_Stacja_elektroenergetyczna_\"Jamki\"_220_110kV"/LConn3 -- 220kV_Byczyna___Jamki_CN_40946790_220000_CN_133537926_220000/RConn3 -- 220kV_Łagisza___Jamki_CN_40946790_220000_CN_66161634_220000/LConn3 -- bus47/LConn1
  220kV_Byczyna___Jamki_CN_40946790_220000_CN_66051759_220000/RConn1 -- "T_66051759__Stacja_elektroenergetyczna_\"Koksochemia\"_220kV"/LConn1 -- 220kV_Koksochemia___Łośnice_CN_66051759_220000_CN_153838553_220000/LConn1 -- 220kV_Koksochemia___Łośnice_CN_66051759_220000_CN_187420591_220000/RConn1
  220kV_Byczyna___Jamki_CN_40946790_220000_CN_66051759_220000/RConn2 -- "T_66051759__Stacja_elektroenergetyczna_\"Koksochemia\"_220kV"/LConn2 -- 220kV_Koksochemia___Łośnice_CN_66051759_220000_CN_153838553_220000/LConn2 -- 220kV_Koksochemia___Łośnice_CN_66051759_220000_CN_187420591_220000/RConn2
  220kV_Byczyna___Jamki_CN_40946790_220000_CN_66051759_220000/RConn3 -- "T_66051759__Stacja_elektroenergetyczna_\"Koksochemia\"_220kV"/LConn3 -- 220kV_Koksochemia___Łośnice_CN_66051759_220000_CN_153838553_220000/LConn3 -- 220kV_Koksochemia___Łośnice_CN_66051759_220000_CN_187420591_220000/RConn3 -- bus48/LConn1
  220kV_Łagisza___Jamki_CN_40946790_220000_CN_66161634_220000/RConn1 -- "T_66161634_400000;220000;110000_Stacja_elektroenergetyczna_\"Łagisza\"_400_220_110_kV"/RConn1 -- 220kV_Blachownia___Łagisza_CN_185454704_220000_CN_66161634_220000/LConn1 -- 220kV_Łagisza___Byczyna___Halemba_CN_133537926_220000_CN_66161634_220000/RConn1 -- 220kV_Joachimów___Huta_Częstochowa_CN_224727316_220000_CN_66161634_220000/LConn1 -- L_66161634/LConn1
  220kV_Łagisza___Jamki_CN_40946790_220000_CN_66161634_220000/RConn2 -- "T_66161634_400000;220000;110000_Stacja_elektroenergetyczna_\"Łagisza\"_400_220_110_kV"/RConn2 -- 220kV_Blachownia___Łagisza_CN_185454704_220000_CN_66161634_220000/LConn2 -- 220kV_Łagisza___Byczyna___Halemba_CN_133537926_220000_CN_66161634_220000/RConn2 -- 220kV_Joachimów___Huta_Częstochowa_CN_224727316_220000_CN_66161634_220000/LConn2 -- L_66161634/LConn2
  220kV_Łagisza___Jamki_CN_40946790_220000_CN_66161634_220000/RConn3 -- "T_66161634_400000;220000;110000_Stacja_elektroenergetyczna_\"Łagisza\"_400_220_110_kV"/RConn3 -- 220kV_Blachownia___Łagisza_CN_185454704_220000_CN_66161634_220000/LConn3 -- 220kV_Łagisza___Byczyna___Halemba_CN_133537926_220000_CN_66161634_220000/RConn3 -- 220kV_Joachimów___Huta_Częstochowa_CN_224727316_220000_CN_66161634_220000/LConn3 -- L_66161634/LConn3 -- bus49/LConn1
  "T_191038569__Stacja_elektroenergetyczna_\"Azoty_Tarnów\"_220_110kV"/LConn1 -- 220kV_Klikowa___Azoty_Tarnów_CN_191038569_220000_CN_191035265_220000/RConn1
  "T_191038569__Stacja_elektroenergetyczna_\"Azoty_Tarnów\"_220_110kV"/LConn2 -- 220kV_Klikowa___Azoty_Tarnów_CN_191038569_220000_CN_191035265_220000/RConn2
  220kV_Klikowa___Azoty_Tarnów_CN_191038569_220000_CN_191035265_220000/RConn3 -- "T_191038569__Stacja_elektroenergetyczna_\"Azoty_Tarnów\"_220_110kV"/LConn3 -- bus50/LConn1
  "T_89434732__Stacja_elektroenergetyczna_\"Towarowa\"_220_110_15kV"/LConn1 -- 220kV_Mory___Towarowa_CN_89434732_220000_CN_29115701_220000/RConn1
  "T_89434732__Stacja_elektroenergetyczna_\"Towarowa\"_220_110_15kV"/LConn2 -- 220kV_Mory___Towarowa_CN_89434732_220000_CN_29115701_220000/RConn2
  220kV_Mory___Towarowa_CN_89434732_220000_CN_29115701_220000/RConn3 -- "T_89434732__Stacja_elektroenergetyczna_\"Towarowa\"_220_110_15kV"/LConn3 -- bus51/LConn1
  220kV_Blachownia___Łagisza_CN_185454704_220000_CN_66161634_220000/RConn1 -- "T_185454704__Stacja_elektroenergetyczna_\"Blachownia\"_220_110kV"/LConn1 -- 220kV_Wielopole___Blachownia_CN_185454704_220000_CN_185459155_220000/LConn1 -- 220kV_Wielopole___Blachownia_CN_185454704_220000_CN_336990960_220000/LConn1 -- 220kV_Wielopole___Blachownia_CN_185454704_220000_CN_139452056_220000/RConn1
  220kV_Blachownia___Łagisza_CN_185454704_220000_CN_66161634_220000/RConn2 -- "T_185454704__Stacja_elektroenergetyczna_\"Blachownia\"_220_110kV"/LConn2 -- 220kV_Wielopole___Blachownia_CN_185454704_220000_CN_185459155_220000/LConn2 -- 220kV_Wielopole___Blachownia_CN_185454704_220000_CN_336990960_220000/LConn2 -- 220kV_Wielopole___Blachownia_CN_185454704_220000_CN_139452056_220000/RConn2
  220kV_Blachownia___Łagisza_CN_185454704_220000_CN_66161634_220000/RConn3 -- "T_185454704__Stacja_elektroenergetyczna_\"Blachownia\"_220_110kV"/LConn3 -- 220kV_Wielopole___Blachownia_CN_185454704_220000_CN_185459155_220000/LConn3 -- 220kV_Wielopole___Blachownia_CN_185454704_220000_CN_336990960_220000/LConn3 -- bus52/LConn1 -- 220kV_Wielopole___Blachownia_CN_185454704_220000_CN_139452056_220000/RConn3
  "T_185459155__Stacja_elektroenergetyczna_\"Kędzierzyn\"_220_110kV"/LConn1 -- 220kV_Wielopole___Blachownia_CN_185454704_220000_CN_185459155_220000/RConn1
  "T_185459155__Stacja_elektroenergetyczna_\"Kędzierzyn\"_220_110kV"/LConn2 -- 220kV_Wielopole___Blachownia_CN_185454704_220000_CN_185459155_220000/RConn2
  220kV_Wielopole___Blachownia_CN_185454704_220000_CN_185459155_220000/RConn3 -- "T_185459155__Stacja_elektroenergetyczna_\"Kędzierzyn\"_220_110kV"/LConn3 -- bus53/LConn1
  220kV_Wielopole___Blachownia_CN_185454704_220000_CN_336990960_220000/RConn1 -- "T_336990960_220000;110000_Stacja_Energetyczna_\"Groszowice\"_220_110_kV"/LConn1 -- 220kV_Ząbkowice___Groszowice_CN_336990960_220000_CN_179279860_220000/LConn1
  220kV_Wielopole___Blachownia_CN_185454704_220000_CN_336990960_220000/RConn2 -- "T_336990960_220000;110000_Stacja_Energetyczna_\"Groszowice\"_220_110_kV"/LConn2 -- 220kV_Ząbkowice___Groszowice_CN_336990960_220000_CN_179279860_220000/LConn2
  220kV_Wielopole___Blachownia_CN_185454704_220000_CN_336990960_220000/RConn3 -- "T_336990960_220000;110000_Stacja_Energetyczna_\"Groszowice\"_220_110_kV"/LConn3 -- 220kV_Ząbkowice___Groszowice_CN_336990960_220000_CN_179279860_220000/LConn3 -- bus54/LConn1
  220kV_Sochaczew___Ołtarzew_CN_251239544_220000_CN_145037309_220000/LConn1 -- "T_251239544_400000;220000;110000_Stacja_elektroenergetyczna_\"Ołtarzew\"_400_220_110kV"/RConn1 -- 220kV_Janów___Ołtarzew_CN_251239544_220000_CN_35366436_220000/RConn1 -- L_251239544/LConn1 -- 220kV_Ołtarzew___Mory_CN_251239544_220000_CN_29115701_220000/RConn1
  220kV_Sochaczew___Ołtarzew_CN_251239544_220000_CN_145037309_220000/LConn2 -- "T_251239544_400000;220000;110000_Stacja_elektroenergetyczna_\"Ołtarzew\"_400_220_110kV"/RConn2 -- 220kV_Janów___Ołtarzew_CN_251239544_220000_CN_35366436_220000/RConn2 -- L_251239544/LConn2 -- 220kV_Ołtarzew___Mory_CN_251239544_220000_CN_29115701_220000/RConn2
  220kV_Sochaczew___Ołtarzew_CN_251239544_220000_CN_145037309_220000/LConn3 -- "T_251239544_400000;220000;110000_Stacja_elektroenergetyczna_\"Ołtarzew\"_400_220_110kV"/RConn3 -- 220kV_Janów___Ołtarzew_CN_251239544_220000_CN_35366436_220000/RConn3 -- L_251239544/LConn3 -- bus55/LConn1 -- 220kV_Ołtarzew___Mory_CN_251239544_220000_CN_29115701_220000/RConn3
  220kV_Sochaczew___Ołtarzew_CN_251239544_220000_CN_145037309_220000/RConn1 -- "T_145037309_220000;110000_Stacja_elektroenergetyczna_\"Sochaczew\"_220_110kV"/LConn1 -- 220kV_Konin___Sochaczew_CN_145037309_220000_CN_216975352_220000/RConn1
  220kV_Sochaczew___Ołtarzew_CN_251239544_220000_CN_145037309_220000/RConn2 -- "T_145037309_220000;110000_Stacja_elektroenergetyczna_\"Sochaczew\"_220_110kV"/LConn2 -- 220kV_Konin___Sochaczew_CN_145037309_220000_CN_216975352_220000/RConn2
  220kV_Sochaczew___Ołtarzew_CN_251239544_220000_CN_145037309_220000/RConn3 -- "T_145037309_220000;110000_Stacja_elektroenergetyczna_\"Sochaczew\"_220_110kV"/LConn3 -- 220kV_Konin___Sochaczew_CN_145037309_220000_CN_216975352_220000/RConn3 -- bus56/LConn1
  "T_216060722_220000;110000_Stacja_elektroenergetyczna_\"Aniołów\"_220_110_kV"/LConn1 -- 220kV_Rogowiec___Joachimów_tor_2_CN_293484891_220000_CN_216060722_220000/RConn1
  "T_216060722_220000;110000_Stacja_elektroenergetyczna_\"Aniołów\"_220_110_kV"/LConn2 -- 220kV_Rogowiec___Joachimów_tor_2_CN_293484891_220000_CN_216060722_220000/RConn2
  220kV_Rogowiec___Joachimów_tor_2_CN_293484891_220000_CN_216060722_220000/RConn3 -- "T_216060722_220000;110000_Stacja_elektroenergetyczna_\"Aniołów\"_220_110_kV"/LConn3 -- bus57/LConn1
  220kV_Rogowiec___Joachimów_tor_2_CN_293484891_220000_CN_241842600_220000/RConn1 -- T_241842600_400000;220000_Stacja_elektroenergetyczna_„Joachimów”_400_220_kV/RConn1 -- 220kV_Joachimów___Huta_Częstochowa_CN_224727316_220000_CN_241842600_220000/LConn1 -- L_241842600/LConn1 -- 220kV_Łośnice___Kielce_CN_199098050_220000_CN_241842600_220000/LConn1
  220kV_Rogowiec___Joachimów_tor_2_CN_293484891_220000_CN_241842600_220000/RConn2 -- T_241842600_400000;220000_Stacja_elektroenergetyczna_„Joachimów”_400_220_kV/RConn2 -- 220kV_Joachimów___Huta_Częstochowa_CN_224727316_220000_CN_241842600_220000/LConn2 -- L_241842600/LConn2 -- 220kV_Łośnice___Kielce_CN_199098050_220000_CN_241842600_220000/LConn2
  220kV_Rogowiec___Joachimów_tor_2_CN_293484891_220000_CN_241842600_220000/RConn3 -- T_241842600_400000;220000_Stacja_elektroenergetyczna_„Joachimów”_400_220_kV/RConn3 -- 220kV_Joachimów___Huta_Częstochowa_CN_224727316_220000_CN_241842600_220000/LConn3 -- L_241842600/LConn3 -- bus58/LConn1 -- 220kV_Łośnice___Kielce_CN_199098050_220000_CN_241842600_220000/LConn3
  "T_148197330_220000;110000_Stacja_elektroenergetyczna_\"Leszno\"_220_110_kV"/LConn1 -- 220kV_Plewiska___Leszno_CN_32036484_220000_CN_148197330_220000/RConn1
  "T_148197330_220000;110000_Stacja_elektroenergetyczna_\"Leszno\"_220_110_kV"/LConn2 -- 220kV_Plewiska___Leszno_CN_32036484_220000_CN_148197330_220000/RConn2
  220kV_Plewiska___Leszno_CN_32036484_220000_CN_148197330_220000/RConn3 -- "T_148197330_220000;110000_Stacja_elektroenergetyczna_\"Leszno\"_220_110_kV"/LConn3 -- bus59/LConn1
  220kV_Plewiska___Piła_Krzewina_CN_32036484_220000_CN_238640596_220000/RConn1 -- "T_238640596_220000;110000_Stacja_elektroenergetyczna_\"Piła_Krzewina\"_220_110_kV"/LConn1 -- 220kV_Piła_Krzewina___Żydowo_CN_178838661_220000_CN_238640596_220000/RConn1
  220kV_Plewiska___Piła_Krzewina_CN_32036484_220000_CN_238640596_220000/RConn2 -- "T_238640596_220000;110000_Stacja_elektroenergetyczna_\"Piła_Krzewina\"_220_110_kV"/LConn2 -- 220kV_Piła_Krzewina___Żydowo_CN_178838661_220000_CN_238640596_220000/RConn2
  220kV_Plewiska___Piła_Krzewina_CN_32036484_220000_CN_238640596_220000/RConn3 -- "T_238640596_220000;110000_Stacja_elektroenergetyczna_\"Piła_Krzewina\"_220_110_kV"/LConn3 -- 220kV_Piła_Krzewina___Żydowo_CN_178838661_220000_CN_238640596_220000/RConn3 -- bus60/LConn1
  220kV_Glinki___Police_CN_165763717_220000_CN_40062974_220000/RConn1 -- "T_40062974_220000;110000_Stacja_elektroenergetyczna_\"Glinki\"_220_110_kV"/LConn1 -- 220kV_Krajnik___Glinki_CN_39428977_220000_CN_40062974_220000/RConn1
  220kV_Glinki___Police_CN_165763717_220000_CN_40062974_220000/RConn2 -- "T_40062974_220000;110000_Stacja_elektroenergetyczna_\"Glinki\"_220_110_kV"/LConn2 -- 220kV_Krajnik___Glinki_CN_39428977_220000_CN_40062974_220000/RConn2
  220kV_Glinki___Police_CN_165763717_220000_CN_40062974_220000/RConn3 -- "T_40062974_220000;110000_Stacja_elektroenergetyczna_\"Glinki\"_220_110_kV"/LConn3 -- 220kV_Krajnik___Glinki_CN_39428977_220000_CN_40062974_220000/RConn3 -- bus61/LConn1
  G_105864304_Elektrownia_Jaworzno_III/RConn1 -- 220kV_BLOK_1___Byczyna_CN_133537926_220000_CN_105864304_220000/RConn1
  G_105864304_Elektrownia_Jaworzno_III/RConn2 -- 220kV_BLOK_1___Byczyna_CN_133537926_220000_CN_105864304_220000/RConn2
  220kV_BLOK_1___Byczyna_CN_133537926_220000_CN_105864304_220000/RConn3 -- G_105864304_Elektrownia_Jaworzno_III/RConn3 -- bus62/LConn1
  "T_183259405__Stacja_elektroenergetyczna_\"Halemba\"_220_110kV"/LConn1 -- 220kV_Łagisza___Byczyna___Halemba_CN_133537926_220000_CN_183259405_220000/RConn1
  "T_183259405__Stacja_elektroenergetyczna_\"Halemba\"_220_110kV"/LConn2 -- 220kV_Łagisza___Byczyna___Halemba_CN_133537926_220000_CN_183259405_220000/RConn2
  220kV_Łagisza___Byczyna___Halemba_CN_133537926_220000_CN_183259405_220000/RConn3 -- "T_183259405__Stacja_elektroenergetyczna_\"Halemba\"_220_110kV"/LConn3 -- bus63/LConn1
  "T_29139402_220000;110000_Stacja_elektroenergetyczna_\"Katowice\"_220_110_kV"/LConn1 -- 220kV_Łagisza___Byczyna___Halemba_CN_133537926_220000_CN_29139402_220000/RConn1
  "T_29139402_220000;110000_Stacja_elektroenergetyczna_\"Katowice\"_220_110_kV"/LConn2 -- 220kV_Łagisza___Byczyna___Halemba_CN_133537926_220000_CN_29139402_220000/RConn2
  220kV_Łagisza___Byczyna___Halemba_CN_133537926_220000_CN_29139402_220000/RConn3 -- "T_29139402_220000;110000_Stacja_elektroenergetyczna_\"Katowice\"_220_110_kV"/LConn3 -- bus64/LConn1
  220kV_Kozienice___Puławy_CN_88544449_220000_CN_173582810_220000/LConn1 -- "T_88544449__Stacja_elektroenergetyczna_\"Puławy\"_220kV"/LConn1 -- 220kV_Rożki___Puławy_CN_88544449_220000_CN_189851841_220000/LConn1 -- 220kV_Puławy___Abramowice_CN_88544449_220000_CN_170249563_220000/LConn1
  220kV_Kozienice___Puławy_CN_88544449_220000_CN_173582810_220000/LConn2 -- "T_88544449__Stacja_elektroenergetyczna_\"Puławy\"_220kV"/LConn2 -- 220kV_Rożki___Puławy_CN_88544449_220000_CN_189851841_220000/LConn2 -- 220kV_Puławy___Abramowice_CN_88544449_220000_CN_170249563_220000/LConn2
  220kV_Kozienice___Puławy_CN_88544449_220000_CN_173582810_220000/LConn3 -- "T_88544449__Stacja_elektroenergetyczna_\"Puławy\"_220kV"/LConn3 -- 220kV_Rożki___Puławy_CN_88544449_220000_CN_189851841_220000/LConn3 -- bus65/LConn1 -- 220kV_Puławy___Abramowice_CN_88544449_220000_CN_170249563_220000/LConn3
  220kV_Kozienice___Puławy_CN_88544449_220000_CN_173582810_220000/RConn1 -- "T_173582810_400000;220000;110000_Stacja_elektroenergetyczna_\"Kozienice\"_400_220_110_kV"/RConn1 -- 220kV_Mory___Piaseczno_CN_29115701_220000_CN_173582810_220000/RConn1 -- 220kV_Kozienice___Rożki_1_CN_173582810_220000_CN_189851841_220000/LConn1 -- L_173582810/LConn1
  220kV_Kozienice___Puławy_CN_88544449_220000_CN_173582810_220000/RConn2 -- "T_173582810_400000;220000;110000_Stacja_elektroenergetyczna_\"Kozienice\"_400_220_110_kV"/RConn2 -- 220kV_Mory___Piaseczno_CN_29115701_220000_CN_173582810_220000/RConn2 -- 220kV_Kozienice___Rożki_1_CN_173582810_220000_CN_189851841_220000/LConn2 -- L_173582810/LConn2
  220kV_Kozienice___Puławy_CN_88544449_220000_CN_173582810_220000/RConn3 -- "T_173582810_400000;220000;110000_Stacja_elektroenergetyczna_\"Kozienice\"_400_220_110_kV"/RConn3 -- 220kV_Mory___Piaseczno_CN_29115701_220000_CN_173582810_220000/RConn3 -- 220kV_Kozienice___Rożki_1_CN_173582810_220000_CN_189851841_220000/LConn3 -- L_173582810/LConn3 -- bus66/LConn1
  220kV_Puławy___Abramowice_CN_88544449_220000_CN_170249563_220000/RConn1 -- "T_170249563_220000;110000_Stacja_elektroenergetyczna_\"Abramowice\"_220_110_kV"/LConn1 -- 220kV_Mokre___Chełm_CN_194903381_220000_CN_170249563_220000/LConn1
  220kV_Puławy___Abramowice_CN_88544449_220000_CN_170249563_220000/RConn2 -- "T_170249563_220000;110000_Stacja_elektroenergetyczna_\"Abramowice\"_220_110_kV"/LConn2 -- 220kV_Mokre___Chełm_CN_194903381_220000_CN_170249563_220000/LConn2
  220kV_Puławy___Abramowice_CN_88544449_220000_CN_170249563_220000/RConn3 -- "T_170249563_220000;110000_Stacja_elektroenergetyczna_\"Abramowice\"_220_110_kV"/LConn3 -- 220kV_Mokre___Chełm_CN_194903381_220000_CN_170249563_220000/LConn3 -- bus67/LConn1
  220kV_Rożki___Puławy_CN_88544449_220000_CN_189851841_220000/RConn1 -- T_189851841_220000;110000_Stacja_elektroenergetyczna_„Rożki”_220_110_kV/LConn1 -- 220kV_Kielce___Rożki_CN_199098050_220000_CN_189851841_220000/LConn1 -- _CN_254235846_220000_CN_189851841_220000/LConn1 -- 220kV_Kozienice___Rożki_1_CN_173582810_220000_CN_189851841_220000/RConn1
  220kV_Rożki___Puławy_CN_88544449_220000_CN_189851841_220000/RConn2 -- T_189851841_220000;110000_Stacja_elektroenergetyczna_„Rożki”_220_110_kV/LConn2 -- 220kV_Kielce___Rożki_CN_199098050_220000_CN_189851841_220000/LConn2 -- _CN_254235846_220000_CN_189851841_220000/LConn2 -- 220kV_Kozienice___Rożki_1_CN_173582810_220000_CN_189851841_220000/RConn2
  220kV_Rożki___Puławy_CN_88544449_220000_CN_189851841_220000/RConn3 -- T_189851841_220000;110000_Stacja_elektroenergetyczna_„Rożki”_220_110_kV/LConn3 -- 220kV_Kielce___Rożki_CN_199098050_220000_CN_189851841_220000/LConn3 -- _CN_254235846_220000_CN_189851841_220000/LConn3 -- 220kV_Kozienice___Rożki_1_CN_173582810_220000_CN_189851841_220000/RConn3 -- bus68/LConn1
  220_kV_Bydgoszcz_Jasiniec___Grudziądz_Węgrowo_CN_46092396_220000_CN_46235456_220000/RConn1 -- "T_46092396_400000;220000;110000_Stacja_elektroenergetyczna_\"Grudziądz___Węgrowo\"_400_220_110_kV"/RConn1 -- 220kV_Toruń_Elana___Grudziądz_Węgrowo_CN_46092396_220000_CN_143484238_220000/LConn1 -- L_46092396/LConn1
  220_kV_Bydgoszcz_Jasiniec___Grudziądz_Węgrowo_CN_46092396_220000_CN_46235456_220000/RConn2 -- "T_46092396_400000;220000;110000_Stacja_elektroenergetyczna_\"Grudziądz___Węgrowo\"_400_220_110_kV"/RConn2 -- 220kV_Toruń_Elana___Grudziądz_Węgrowo_CN_46092396_220000_CN_143484238_220000/LConn2 -- L_46092396/LConn2
  220_kV_Bydgoszcz_Jasiniec___Grudziądz_Węgrowo_CN_46092396_220000_CN_46235456_220000/RConn3 -- "T_46092396_400000;220000;110000_Stacja_elektroenergetyczna_\"Grudziądz___Węgrowo\"_400_220_110_kV"/RConn3 -- 220kV_Toruń_Elana___Grudziądz_Węgrowo_CN_46092396_220000_CN_143484238_220000/LConn3 -- L_46092396/LConn3 -- bus69/LConn1
  220kV_Toruń_Elana___Grudziądz_Węgrowo_CN_46092396_220000_CN_143484238_220000/RConn1 -- T_143484238_220000;110000_Stacja_elektroenergetyczna_„Toruń___Elana”_220_110_kV/LConn1 -- 220kV_Toruń_Elana___Włocławek_Azoty_CN_72879943_220000_CN_143484238_220000/RConn1
  220kV_Toruń_Elana___Grudziądz_Węgrowo_CN_46092396_220000_CN_143484238_220000/RConn2 -- T_143484238_220000;110000_Stacja_elektroenergetyczna_„Toruń___Elana”_220_110_kV/LConn2 -- 220kV_Toruń_Elana___Włocławek_Azoty_CN_72879943_220000_CN_143484238_220000/RConn2
  220kV_Toruń_Elana___Grudziądz_Węgrowo_CN_46092396_220000_CN_143484238_220000/RConn3 -- T_143484238_220000;110000_Stacja_elektroenergetyczna_„Toruń___Elana”_220_110_kV/LConn3 -- 220kV_Toruń_Elana___Włocławek_Azoty_CN_72879943_220000_CN_143484238_220000/RConn3 -- bus70/LConn1
  220kV_Ostrołęka_2___Olsztyn_CN_101915790_220000_CN_121656686_220000/LConn1 -- T_101915790_220000;110000;15000_Stacja_elektroenergetyczna_„Olsztyn_I”_220_110_15_kV/LConn1 -- 220kV_Olsztyn_I___Olsztyn_Mątki_CN_101915790_220000_CN_101914781_220000/LConn1 -- 220kV_Włocławek___Olsztyn_CN_101915790_220000_CN_72879943_220000/RConn1
  220kV_Ostrołęka_2___Olsztyn_CN_101915790_220000_CN_121656686_220000/LConn2 -- T_101915790_220000;110000;15000_Stacja_elektroenergetyczna_„Olsztyn_I”_220_110_15_kV/LConn2 -- 220kV_Olsztyn_I___Olsztyn_Mątki_CN_101915790_220000_CN_101914781_220000/LConn2 -- 220kV_Włocławek___Olsztyn_CN_101915790_220000_CN_72879943_220000/RConn2
  220kV_Ostrołęka_2___Olsztyn_CN_101915790_220000_CN_121656686_220000/LConn3 -- T_101915790_220000;110000;15000_Stacja_elektroenergetyczna_„Olsztyn_I”_220_110_15_kV/LConn3 -- 220kV_Olsztyn_I___Olsztyn_Mątki_CN_101915790_220000_CN_101914781_220000/LConn3 -- 220kV_Włocławek___Olsztyn_CN_101915790_220000_CN_72879943_220000/RConn3 -- bus71/LConn1
  220kV_Ostrołęka_2___Olsztyn_CN_101915790_220000_CN_121656686_220000/RConn1 -- "T_121656686_400000;220000;110000_Stacja_elektroenergetyczna_400_220_110kV_\"Ostrołęka\""/RConn1 -- _CN_121656686_220000_CN_97648143_220000/LConn1 -- 220kV_Miłosna___Ostrołęka_CN_121656686_220000_CN_99593626_220000/LConn1 -- 220kV_Ostrołęka___Ełk_CN_121656686_220000_CN_170259740_220000/LConn1 -- L_121656686/LConn1
  220kV_Ostrołęka_2___Olsztyn_CN_101915790_220000_CN_121656686_220000/RConn2 -- "T_121656686_400000;220000;110000_Stacja_elektroenergetyczna_400_220_110kV_\"Ostrołęka\""/RConn2 -- _CN_121656686_220000_CN_97648143_220000/LConn2 -- 220kV_Miłosna___Ostrołęka_CN_121656686_220000_CN_99593626_220000/LConn2 -- 220kV_Ostrołęka___Ełk_CN_121656686_220000_CN_170259740_220000/LConn2 -- L_121656686/LConn2
  220kV_Ostrołęka_2___Olsztyn_CN_101915790_220000_CN_121656686_220000/RConn3 -- "T_121656686_400000;220000;110000_Stacja_elektroenergetyczna_400_220_110kV_\"Ostrołęka\""/RConn3 -- _CN_121656686_220000_CN_97648143_220000/LConn3 -- 220kV_Miłosna___Ostrołęka_CN_121656686_220000_CN_99593626_220000/LConn3 -- 220kV_Ostrołęka___Ełk_CN_121656686_220000_CN_170259740_220000/LConn3 -- L_121656686/LConn3 -- bus72/LConn1
  220kV_Olsztyn_I___Olsztyn_Mątki_CN_101915790_220000_CN_101914781_220000/RConn1 -- T_101914781_400000;220000;110000_Stacja_elektroenergetyczna_„Olsztyn_Mątki”_400_220_110_kV/RConn1 -- L_101914781/LConn1
  220kV_Olsztyn_I___Olsztyn_Mątki_CN_101915790_220000_CN_101914781_220000/RConn2 -- T_101914781_400000;220000;110000_Stacja_elektroenergetyczna_„Olsztyn_Mątki”_400_220_110_kV/RConn2 -- L_101914781/LConn2
  220kV_Olsztyn_I___Olsztyn_Mątki_CN_101915790_220000_CN_101914781_220000/RConn3 -- T_101914781_400000;220000;110000_Stacja_elektroenergetyczna_„Olsztyn_Mątki”_400_220_110_kV/RConn3 -- L_101914781/LConn3 -- bus73/LConn1
  G_97648143_Elektrownie_Ostrołęka/RConn1 -- _CN_121656686_220000_CN_97648143_220000/RConn1
  G_97648143_Elektrownie_Ostrołęka/RConn2 -- _CN_121656686_220000_CN_97648143_220000/RConn2
  _CN_121656686_220000_CN_97648143_220000/RConn3 -- G_97648143_Elektrownie_Ostrołęka/RConn3 -- bus74/LConn1
  220kV_Miłosna___Ostrołęka_CN_121656686_220000_CN_99593626_220000/RConn1 -- "T_99593626_400000;220000;110000_Stacja_elektroenergetyczna_\"Miłosna\"_400_220_110_kV"/RConn1 -- 220_kV_Mory___Miłosna_CN_29115701_220000_CN_99593626_220000/RConn1 -- L_99593626/LConn1
  220kV_Miłosna___Ostrołęka_CN_121656686_220000_CN_99593626_220000/RConn2 -- "T_99593626_400000;220000;110000_Stacja_elektroenergetyczna_\"Miłosna\"_400_220_110_kV"/RConn2 -- 220_kV_Mory___Miłosna_CN_29115701_220000_CN_99593626_220000/RConn2 -- L_99593626/LConn2
  220kV_Miłosna___Ostrołęka_CN_121656686_220000_CN_99593626_220000/RConn3 -- "T_99593626_400000;220000;110000_Stacja_elektroenergetyczna_\"Miłosna\"_400_220_110_kV"/RConn3 -- 220_kV_Mory___Miłosna_CN_29115701_220000_CN_99593626_220000/RConn3 -- L_99593626/LConn3 -- bus75/LConn1
  "T_170259740_220000;110000_Stacja_elektroenergetyczna_\"Ełk\"_220_110_kV"/LConn1 -- 220kV_Ostrołęka___Ełk_CN_121656686_220000_CN_170259740_220000/RConn1
  "T_170259740_220000;110000_Stacja_elektroenergetyczna_\"Ełk\"_220_110_kV"/LConn2 -- 220kV_Ostrołęka___Ełk_CN_121656686_220000_CN_170259740_220000/RConn2
  220kV_Ostrołęka___Ełk_CN_121656686_220000_CN_170259740_220000/RConn3 -- "T_170259740_220000;110000_Stacja_elektroenergetyczna_\"Ełk\"_220_110_kV"/LConn3 -- bus76/LConn1
  220kV_Mikułowa___Cieplice_CN_178756295_220000_CN_111615226_220000/LConn1 -- "T_178756295_220000;110000_Stacja_elektroenergetyczna_\"Cieplice\"_220_110_kV"/LConn1 -- 220kV_Cieplice___Boguszów_CN_178756295_220000_CN_177749653_220000/LConn1
  220kV_Mikułowa___Cieplice_CN_178756295_220000_CN_111615226_220000/LConn2 -- "T_178756295_220000;110000_Stacja_elektroenergetyczna_\"Cieplice\"_220_110_kV"/LConn2 -- 220kV_Cieplice___Boguszów_CN_178756295_220000_CN_177749653_220000/LConn2
  220kV_Mikułowa___Cieplice_CN_178756295_220000_CN_111615226_220000/LConn3 -- "T_178756295_220000;110000_Stacja_elektroenergetyczna_\"Cieplice\"_220_110_kV"/LConn3 -- 220kV_Cieplice___Boguszów_CN_178756295_220000_CN_177749653_220000/LConn3 -- bus77/LConn1
  220kV_Mikułowa___Cieplice_CN_178756295_220000_CN_111615226_220000/RConn1 -- T_111615226_400000;220000;110000_Stacja_elektroenergetyczna_„Mikułowa”_400_220_110_kV/RConn1 -- 220kV_Mikułowa___Polkowice_CN_180542657_220000_CN_111615226_220000/RConn1 -- 220kV_Mikułowa___Swiebodzice_CN_111615226_220000_CN_179138441_220000/RConn1 -- 220kV_Turów___Mikułowa_CN_111615226_220000_CN_90038401_220000/LConn1 -- 220kV_Mikułowa___Leśniów_CN_111615226_220000_CN_158232924_220000/RConn1 -- L_111615226/LConn1
  220kV_Mikułowa___Cieplice_CN_178756295_220000_CN_111615226_220000/RConn2 -- T_111615226_400000;220000;110000_Stacja_elektroenergetyczna_„Mikułowa”_400_220_110_kV/RConn2 -- 220kV_Mikułowa___Polkowice_CN_180542657_220000_CN_111615226_220000/RConn2 -- 220kV_Mikułowa___Swiebodzice_CN_111615226_220000_CN_179138441_220000/RConn2 -- 220kV_Turów___Mikułowa_CN_111615226_220000_CN_90038401_220000/LConn2 -- 220kV_Mikułowa___Leśniów_CN_111615226_220000_CN_158232924_220000/RConn2 -- L_111615226/LConn2
  220kV_Mikułowa___Cieplice_CN_178756295_220000_CN_111615226_220000/RConn3 -- T_111615226_400000;220000;110000_Stacja_elektroenergetyczna_„Mikułowa”_400_220_110_kV/RConn3 -- 220kV_Mikułowa___Polkowice_CN_180542657_220000_CN_111615226_220000/RConn3 -- 220kV_Mikułowa___Swiebodzice_CN_111615226_220000_CN_179138441_220000/RConn3 -- 220kV_Turów___Mikułowa_CN_111615226_220000_CN_90038401_220000/LConn3 -- 220kV_Mikułowa___Leśniów_CN_111615226_220000_CN_158232924_220000/RConn3 -- L_111615226/LConn3 -- bus78/LConn1
  220kV_Cieplice___Boguszów_CN_178756295_220000_CN_177749653_220000/RConn1 -- "T_177749653_220000;110000_Stacja_elektroenergetyczna_\"Boguszów\"_220_110_kV"/LConn1 -- 220kV_Boguszów___Świebodzice_CN_177749653_220000_CN_179138441_220000/RConn1
  220kV_Cieplice___Boguszów_CN_178756295_220000_CN_177749653_220000/RConn2 -- "T_177749653_220000;110000_Stacja_elektroenergetyczna_\"Boguszów\"_220_110_kV"/LConn2 -- 220kV_Boguszów___Świebodzice_CN_177749653_220000_CN_179138441_220000/RConn2
  220kV_Cieplice___Boguszów_CN_178756295_220000_CN_177749653_220000/RConn3 -- "T_177749653_220000;110000_Stacja_elektroenergetyczna_\"Boguszów\"_220_110_kV"/LConn3 -- 220kV_Boguszów___Świebodzice_CN_177749653_220000_CN_179138441_220000/RConn3 -- bus79/LConn1
  220kV_Koksochemia___Łośnice_CN_66051759_220000_CN_153838553_220000/RConn1 -- T_153838553_220000;110000_Stacja_elektroenergetyczna_„Łośnice”_220_110kV/LConn1 -- 220kV_Łośnice___Kielce_CN_199098050_220000_CN_153838553_220000/LConn1 -- _CN_240806770_220000_CN_153838553_220000/LConn1
  220kV_Koksochemia___Łośnice_CN_66051759_220000_CN_153838553_220000/RConn2 -- T_153838553_220000;110000_Stacja_elektroenergetyczna_„Łośnice”_220_110kV/LConn2 -- 220kV_Łośnice___Kielce_CN_199098050_220000_CN_153838553_220000/LConn2 -- _CN_240806770_220000_CN_153838553_220000/LConn2
  220kV_Koksochemia___Łośnice_CN_66051759_220000_CN_153838553_220000/RConn3 -- T_153838553_220000;110000_Stacja_elektroenergetyczna_„Łośnice”_220_110kV/LConn3 -- 220kV_Łośnice___Kielce_CN_199098050_220000_CN_153838553_220000/LConn3 -- _CN_240806770_220000_CN_153838553_220000/LConn3 -- bus80/LConn1
  "T_248088256__Stacja_elektroenergetyczna_\"Stalowa_Wola\"_220_110_kV"/LConn1 -- 220_kV_Chmielów___Abramowice_odg__Stalowa_Wola_CN_248088256_220000_CN_191352746_220000/LConn1
  "T_248088256__Stacja_elektroenergetyczna_\"Stalowa_Wola\"_220_110_kV"/LConn2 -- 220_kV_Chmielów___Abramowice_odg__Stalowa_Wola_CN_248088256_220000_CN_191352746_220000/LConn2
  220_kV_Chmielów___Abramowice_odg__Stalowa_Wola_CN_248088256_220000_CN_191352746_220000/LConn3 -- "T_248088256__Stacja_elektroenergetyczna_\"Stalowa_Wola\"_220_110_kV"/LConn3 -- bus81/LConn1
  220_kV_Chmielów___Abramowice_odg__Stalowa_Wola_CN_248088256_220000_CN_191352746_220000/RConn1 -- "T_191352746_220000;110000_Stacja_elektroenergetyczna_\"Chmielów\"_220_110_kV"/LConn1 -- 220_kV_Połaniec___Chmielów_CN_199098053_220000_CN_191352746_220000/LConn1 -- 220_kV_Chmielów___Boguchwała_CN_191352746_220000_CN_198635989_220000/LConn1
  220_kV_Chmielów___Abramowice_odg__Stalowa_Wola_CN_248088256_220000_CN_191352746_220000/RConn2 -- "T_191352746_220000;110000_Stacja_elektroenergetyczna_\"Chmielów\"_220_110_kV"/LConn2 -- 220_kV_Połaniec___Chmielów_CN_199098053_220000_CN_191352746_220000/LConn2 -- 220_kV_Chmielów___Boguchwała_CN_191352746_220000_CN_198635989_220000/LConn2
  220_kV_Chmielów___Abramowice_odg__Stalowa_Wola_CN_248088256_220000_CN_191352746_220000/RConn3 -- "T_191352746_220000;110000_Stacja_elektroenergetyczna_\"Chmielów\"_220_110_kV"/LConn3 -- 220_kV_Połaniec___Chmielów_CN_199098053_220000_CN_191352746_220000/LConn3 -- 220_kV_Chmielów___Boguchwała_CN_191352746_220000_CN_198635989_220000/LConn3 -- bus82/LConn1
  220kV_Łośnice___Kielce_CN_199098050_220000_CN_241842600_220000/RConn1 -- "T_199098050_400000;220000_Stacja_elektroenergetyczna_\"Kielce\"_400_220kV"/RConn1 -- 220kV_Kielce___Kielce_Piaski_CN_199098050_220000_CN_228154083_220000/LConn1 -- 220kV_Kielce___Rożki_CN_199098050_220000_CN_189851841_220000/RConn1 -- 220_kV_Kielce___Radkowice_CN_199098050_220000_CN_199098055_220000/LConn1 -- L_199098050/LConn1 -- 220kV_Łośnice___Kielce_CN_199098050_220000_CN_153838553_220000/RConn1
  220kV_Łośnice___Kielce_CN_199098050_220000_CN_241842600_220000/RConn2 -- "T_199098050_400000;220000_Stacja_elektroenergetyczna_\"Kielce\"_400_220kV"/RConn2 -- 220kV_Kielce___Kielce_Piaski_CN_199098050_220000_CN_228154083_220000/LConn2 -- 220kV_Kielce___Rożki_CN_199098050_220000_CN_189851841_220000/RConn2 -- 220_kV_Kielce___Radkowice_CN_199098050_220000_CN_199098055_220000/LConn2 -- L_199098050/LConn2 -- 220kV_Łośnice___Kielce_CN_199098050_220000_CN_153838553_220000/RConn2
  220kV_Łośnice___Kielce_CN_199098050_220000_CN_241842600_220000/RConn3 -- "T_199098050_400000;220000_Stacja_elektroenergetyczna_\"Kielce\"_400_220kV"/RConn3 -- 220kV_Kielce___Kielce_Piaski_CN_199098050_220000_CN_228154083_220000/LConn3 -- 220kV_Kielce___Rożki_CN_199098050_220000_CN_189851841_220000/RConn3 -- 220_kV_Kielce___Radkowice_CN_199098050_220000_CN_199098055_220000/LConn3 -- L_199098050/LConn3 -- bus83/LConn1 -- 220kV_Łośnice___Kielce_CN_199098050_220000_CN_153838553_220000/RConn3
  "T_228154083_220000;110000_Stacja_elektroenergetyczna_\"KIELCE_PIASKI\"_220_110_30_15kV"/LConn1 -- 220kV_Kielce___Kielce_Piaski_CN_199098050_220000_CN_228154083_220000/RConn1
  "T_228154083_220000;110000_Stacja_elektroenergetyczna_\"KIELCE_PIASKI\"_220_110_30_15kV"/LConn2 -- 220kV_Kielce___Kielce_Piaski_CN_199098050_220000_CN_228154083_220000/RConn2
  220kV_Kielce___Kielce_Piaski_CN_199098050_220000_CN_228154083_220000/RConn3 -- "T_228154083_220000;110000_Stacja_elektroenergetyczna_\"KIELCE_PIASKI\"_220_110_30_15kV"/LConn3 -- bus84/LConn1
  220_kV_Kielce___Radkowice_CN_199098050_220000_CN_199098055_220000/RConn1 -- "T_199098055_220000;110000_Stacja_elektroenergetyczna_\"Radkowice\"_220_110_30_15kV"/LConn1 -- 220_kV_Połaniec___Radkowice_CN_199098053_220000_CN_199098055_220000/LConn1
  220_kV_Kielce___Radkowice_CN_199098050_220000_CN_199098055_220000/RConn2 -- "T_199098055_220000;110000_Stacja_elektroenergetyczna_\"Radkowice\"_220_110_30_15kV"/LConn2 -- 220_kV_Połaniec___Radkowice_CN_199098053_220000_CN_199098055_220000/LConn2
  220_kV_Kielce___Radkowice_CN_199098050_220000_CN_199098055_220000/RConn3 -- "T_199098055_220000;110000_Stacja_elektroenergetyczna_\"Radkowice\"_220_110_30_15kV"/LConn3 -- 220_kV_Połaniec___Radkowice_CN_199098053_220000_CN_199098055_220000/LConn3 -- bus85/LConn1
